simulink model "Thruster_Example_rw"  (R2024b)
settings: Solver=ode4  StartTime=0.0  StopTime=2000  FixedStep=0.01  RelTol=1e-3
undefined symbols (not defined in the file): Cube_L, dt, F_vec, Iws, M_rw, m_tot, norm_Ib, Omega1_init, Omega2_init, Omega3_init, Omega4_init, qb0, rad2rpm, RCS_F, RCS_F_vec, RCS_Pos, RCS_pos, RCS_PWM_Freq, RCS_Sampling_time, RCS_THR_vec, REL_TS_POS_I_0, REL_TS_VEL_I_0, RW_As, RW_Max_Speed, RW_Omegad_max, sat, SC_Ib, SC_state0, SS_Total_Mass, TC_Kepler, THR_dt, THR_Force, THR_freq, THR_Pos, TS_Ib, TS_qb0, TS_state0, TS_wb0, wb0, X, Y, Z
libraries: sm_lib x348, nesl_utility x236, simulink_extras x115, sharedtransform x64, aerolibutil x38, simulink x28, sharedutil x13
(part 4 of 16)

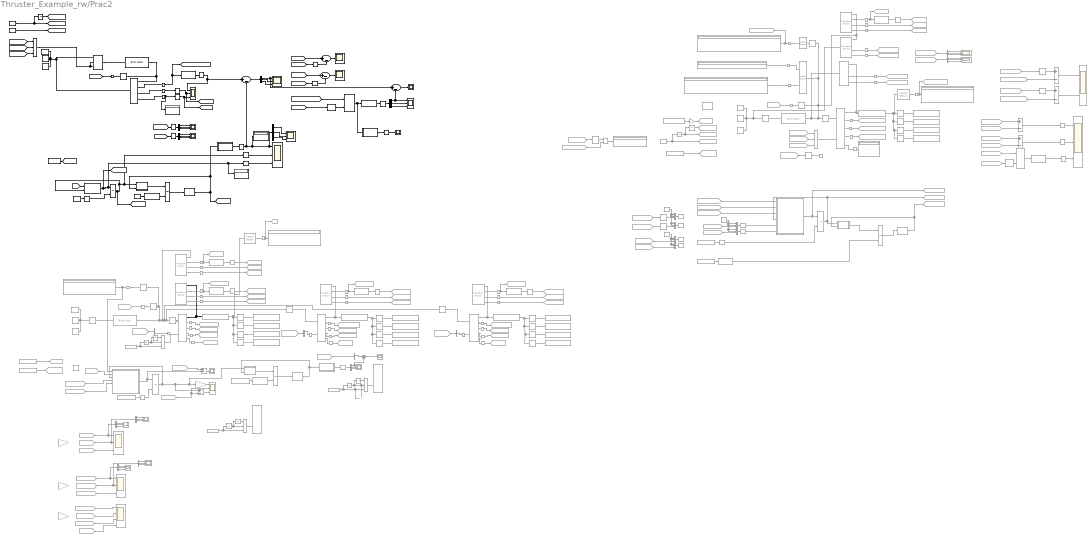
== system Thruster_Example_rw/Prac2 ==
  note: inertia sensor 써야 wheel까지 포함한 MOI 구해짐.
      | 여기서 구해진 MOI를 사용해야 오차가 없다.
  note: 이렇게 하면, wheel의 각가속도, 각속도 다 계산 안해도 넣어진다.
  (rad/sec) to RPM{,1,3..4} (4 alike) : Gain  Commented=on  Gain=60/(2*pi)
  6-DOF Joint : sm_lib/Joints/6-DOF Joint  Commented=on  JointMode=Normal  SenseConstraintForce=off  SenseConstraintForceX=off  SenseConstraintForceY=off  SenseConstraintForceZ=off  SenseConstraintTorque=off  SenseConstraintTorqueX=off  SenseConstraintTorqueY=off  SenseConstraintTorqueZ=off  SenseTotalForce=off  SenseTotalForceX=off  SenseTotalForceY=off  SenseTotalForceZ=off  SenseTotalTorque=off  SenseTotalTorqueX=off  SenseTotalTorqueY=off  SenseTotalTorqueZ=off  CompositeWrenchDir=FollowerOnBase  CompositeWrenchFrame=BaseFrame  PxEquilibriumPosition=0  PxEquilibriumPositionUnits=m  PxSpringStiffness=0  PxSpringStiffnessUnits=N/m  PxDampingCoefficient=0  PxDampingCoefficientUnits=N/(m/s)  PxTorqueActuationMode=NoTorque  PxMotionActuationMode=ComputedMotion  PxSensePosition=off  PxSenseVelocity=off  PxSenseAcceleration=off  PxSenseTorqueForce=off  PxSenseLowerLimitTorqueForce=off  PxSenseUpperLimitTorqueForce=off  PxLowerLimitSpecify=off  PxLowerLimitBound=-1  PxLowerLimitBoundUnits=m  PxLowerLimitStiffness=1e6  PxLowerLimitStiffnessUnits=N/m  PxLowerLimitDamping=1e3  PxLowerLimitDampingUnits=N/(m/s)  PxLowerLimitTransitionRegionWidth=1e-4  PxLowerLimitTransitionRegionWidthUnits=m  PxUpperLimitSpecify=off  PxUpperLimitBound=1  PxUpperLimitBoundUnits=m  PxUpperLimitStiffness=1e6  PxUpperLimitStiffnessUnits=N/m  PxUpperLimitDamping=1e3  PxUpperLimitDampingUnits=N/(m/s)  PxUpperLimitTransitionRegionWidth=1e-4  PxUpperLimitTransitionRegionWidthUnits=m  PxPositionTargetSpecify=off  PxPositionTargetPriority=High  PxPositionTargetValue=0  PxPositionTargetValueUnits=m  PxVelocityTargetSpecify=off  PxVelocityTargetPriority=High  PxVelocityTargetValue=0  PxVelocityTargetValueUnits=m/s  PyEquilibriumPosition=0  PyEquilibriumPositionUnits=m  PySpringStiffness=0  PySpringStiffnessUnits=N/m  PyDampingCoefficient=0  PyDampingCoefficientUnits=N/(m/s)  PyTorqueActuationMode=NoTorque  PyMotionActuationMode=ComputedMotion  PySensePosition=off  PySenseVelocity=off  PySenseAcceleration=off  PySenseTorqueForce=off  PySenseLowerLimitTorqueForce=off  PySenseUpperLimitTorqueForce=off  PyLowerLimitSpecify=off  PyLowerLimitBound=-1  PyLowerLimitBoundUnits=m  PyLowerLimitStiffness=1e6  PyLowerLimitStiffnessUnits=N/m  PyLowerLimitDamping=1e3  PyLowerLimitDampingUnits=N/(m/s)  PyLowerLimitTransitionRegionWidth=1e-4  PyLowerLimitTransitionRegionWidthUnits=m  PyUpperLimitSpecify=off  PyUpperLimitBound=1  PyUpperLimitBoundUnits=m  PyUpperLimitStiffness=1e6  PyUpperLimitStiffnessUnits=N/m  PyUpperLimitDamping=1e3  PyUpperLimitDampingUnits=N/(m/s)  PyUpperLimitTransitionRegionWidth=1e-4  PyUpperLimitTransitionRegionWidthUnits=m  PyPositionTargetSpecify=off  PyPositionTargetPriority=High  PyPositionTargetValue=0  PyPositionTargetValueUnits=m  PyVelocityTargetSpecify=off  PyVelocityTargetPriority=High  PyVelocityTargetValue=0  PyVelocityTargetValueUnits=m/s  PzEquilibriumPosition=0  PzEquilibriumPositionUnits=m  PzSpringStiffness=0  PzSpringStiffnessUnits=N/m  PzDampingCoefficient=0  PzDampingCoefficientUnits=N/(m/s)  PzTorqueActuationMode=NoTorque  PzMotionActuationMode=ComputedMotion  PzSensePosition=off  PzSenseVelocity=off  PzSenseAcceleration=off  PzSenseTorqueForce=off  PzSenseLowerLimitTorqueForce=off  PzSenseUpperLimitTorqueForce=off  PzLowerLimitSpecify=off  PzLowerLimitBound=-1  PzLowerLimitBoundUnits=m  PzLowerLimitStiffness=1e6  PzLowerLimitStiffnessUnits=N/m  PzLowerLimitDamping=1e3  PzLowerLimitDampingUnits=N/(m/s)  PzLowerLimitTransitionRegionWidth=1e-4  PzLowerLimitTransitionRegionWidthUnits=m  PzUpperLimitSpecify=off  PzUpperLimitBound=1  PzUpperLimitBoundUnits=m  PzUpperLimitStiffness=1e6  PzUpperLimitStiffnessUnits=N/m  PzUpperLimitDamping=1e3  PzUpperLimitDampingUnits=N/(m/s)  PzUpperLimitTransitionRegionWidth=1e-4  PzUpperLimitTransitionRegionWidthUnits=m  PzPositionTargetSpecify=off  PzPositionTargetPriority=High  PzPositionTargetValue=0  PzPositionTargetValueUnits=m  PzVelocityTargetSpecify=off  PzVelocityTargetPriority=High  PzVelocityTargetValue=0  PzVelocityTargetValueUnits=m/s  SphEqPosRotationMethod=None  SphEqPosRotationAngleUnits=deg  SphEqPosRotationStandardAxis=+Z  SphEqPosRotationAngle=0.0  SphEqPosRotationArbitraryAxis=[0 0 1]  SphEqPosFollAlignAxisA=+X  SphEqPosBaseAlignAxisA=+Y  SphEqPosFollAlignAxisB=+Y  SphEqPosBaseAlignAxisB=+Z  SphEqPosRotationSequenceAxes=FollowerAxes  SphEqPosRotationSequence=XYX  SphEqPosRotationSequenceAngles=[0 0 0]  SphEqPosRotationSequenceAnglesUnits=deg  SphEqPosRotationMatrix=[1 0 0; 0 1 0; 0 0 1]  SphEqPosQuaternion=[1 0 0 0]  SphSpringStiffness=0  SphSpringStiffnessUnits=N*m/deg  SphDampingCoefficient=0  SphDampingCoefficientUnits=N*m/(deg/s)  SphActuateTorqueX=off  SphActuateTorqueY=off  SphActuateTorqueZ=on  SphActuateTorque=off  SphTorqueActuationMode=NoTorque  SphMotionActuationMode=ComputedMotion  SphActuationFrame=BaseFrame  SphSensePosition=off  SphSenseVelocityX=off  SphSenseVelocityY=off  SphSenseVelocityZ=off  SphSenseVelocity=off  SphSenseAccelerationX=off  SphSenseAccelerationY=off  SphSenseAccelerationZ=off  SphSenseAcceleration=off  SphSenseTorqueX=off  SphSenseTorqueY=off  SphSenseTorqueZ=off  SphSenseTorqueForce=off  SphSenseLowerLimitTorqueMag=off  SphSenseUpperLimitTorqueMag=off  SphSensingFrame=BaseFrame  SphLowerLimitSpecify=off  SphLowerLimitBound=15  SphLowerLimitBoundUnits=deg  SphLowerLimitStiffness=1e4  SphLowerLimitStiffnessUnits=N*m/deg  SphLowerLimitDamping=10  SphLowerLimitDampingUnits=N*m/(deg/s)  SphLowerLimitTransitionRegionWidth=0.1  SphLowerLimitTransitionRegionWidthUnits=deg  SphUpperLimitSpecify=off  SphUpperLimitBound=45  SphUpperLimitBoundUnits=deg  SphUpperLimitStiffness=1e4  SphUpperLimitStiffnessUnits=N*m/deg  SphUpperLimitDamping=10  SphUpperLimitDampingUnits=N*m/(deg/s)  SphUpperLimitTransitionRegionWidth=0.1  SphUpperLimitTransitionRegionWidthUnits=deg  SphPositionTargetRotationMethod=None  SphPositionTargetRotationAngleUnits=deg  SphPositionTargetRotationStandardAxis=+Z  SphPositionTargetRotationAngle=0.0  SphPositionTargetRotationArbitraryAxis=[0 0 1]  SphPositionTargetFollAlignAxisA=+X  SphPositionTargetBaseAlignAxisA=+Y  SphPositionTargetFollAlignAxisB=+Y  SphPositionTargetBaseAlignAxisB=+Z  SphPositionTargetRotationSequenceAxes=FollowerAxes  SphPositionTargetRotationSequence=XYX  SphPositionTargetRotationSequenceAngles=[0 0 0]  SphPositionTargetRotationSequenceAnglesUnits=deg  SphPositionTargetRotationMatrix=[1 0 0; 0 1 0; 0 0 1]  SphPositionTargetQuaternion=[1 0 0 0]  SphPositionTargetSpecify=off  SphPositionTargetPriority=High  SphVelocityTargetValue=[0 0 0]  SphVelocityTargetValueUnits=deg/s  SphVelocityTargetSpecify=off  SphVelocityTargetPriority=High  SphVelocityTargetInFollowerFrame=on
  6-DOF Joint2 : sm_lib/Joints/6-DOF Joint  Commented=on  JointMode=Normal  SenseConstraintForce=off  SenseConstraintForceX=off  SenseConstraintForceY=off  SenseConstraintForceZ=off  SenseConstraintTorque=off  SenseConstraintTorqueX=off  SenseConstraintTorqueY=off  SenseConstraintTorqueZ=off  SenseTotalForce=off  SenseTotalForceX=off  SenseTotalForceY=off  SenseTotalForceZ=off  SenseTotalTorque=off  SenseTotalTorqueX=off  SenseTotalTorqueY=off  SenseTotalTorqueZ=off  CompositeWrenchDir=FollowerOnBase  CompositeWrenchFrame=BaseFrame  PxEquilibriumPosition=0  PxEquilibriumPositionUnits=m  PxSpringStiffness=0  PxSpringStiffnessUnits=N/m  PxDampingCoefficient=0  PxDampingCoefficientUnits=N/(m/s)  PxTorqueActuationMode=NoTorque  PxMotionActuationMode=ComputedMotion  PxSensePosition=off  PxSenseVelocity=off  PxSenseAcceleration=off  PxSenseTorqueForce=off  PxSenseLowerLimitTorqueForce=off  PxSenseUpperLimitTorqueForce=off  PxLowerLimitSpecify=off  PxLowerLimitBound=-1  PxLowerLimitBoundUnits=m  PxLowerLimitStiffness=1e6  PxLowerLimitStiffnessUnits=N/m  PxLowerLimitDamping=1e3  PxLowerLimitDampingUnits=N/(m/s)  PxLowerLimitTransitionRegionWidth=1e-4  PxLowerLimitTransitionRegionWidthUnits=m  PxUpperLimitSpecify=off  PxUpperLimitBound=1  PxUpperLimitBoundUnits=m  PxUpperLimitStiffness=1e6  PxUpperLimitStiffnessUnits=N/m  PxUpperLimitDamping=1e3  PxUpperLimitDampingUnits=N/(m/s)  PxUpperLimitTransitionRegionWidth=1e-4  PxUpperLimitTransitionRegionWidthUnits=m  PxPositionTargetSpecify=off  PxPositionTargetPriority=High  PxPositionTargetValue=0  PxPositionTargetValueUnits=m  PxVelocityTargetSpecify=off  PxVelocityTargetPriority=High  PxVelocityTargetValue=0  PxVelocityTargetValueUnits=m/s  PyEquilibriumPosition=0  PyEquilibriumPositionUnits=m  PySpringStiffness=0  PySpringStiffnessUnits=N/m  PyDampingCoefficient=0  PyDampingCoefficientUnits=N/(m/s)  PyTorqueActuationMode=NoTorque  PyMotionActuationMode=ComputedMotion  PySensePosition=off  PySenseVelocity=off  PySenseAcceleration=off  PySenseTorqueForce=off  PySenseLowerLimitTorqueForce=off  PySenseUpperLimitTorqueForce=off  PyLowerLimitSpecify=off  PyLowerLimitBound=-1  PyLowerLimitBoundUnits=m  PyLowerLimitStiffness=1e6  PyLowerLimitStiffnessUnits=N/m  PyLowerLimitDamping=1e3  PyLowerLimitDampingUnits=N/(m/s)  PyLowerLimitTransitionRegionWidth=1e-4  PyLowerLimitTransitionRegionWidthUnits=m  PyUpperLimitSpecify=off  PyUpperLimitBound=1  PyUpperLimitBoundUnits=m  PyUpperLimitStiffness=1e6  PyUpperLimitStiffnessUnits=N/m  PyUpperLimitDamping=1e3  PyUpperLimitDampingUnits=N/(m/s)  PyUpperLimitTransitionRegionWidth=1e-4  PyUpperLimitTransitionRegionWidthUnits=m  PyPositionTargetSpecify=off  PyPositionTargetPriority=High  PyPositionTargetValue=0  PyPositionTargetValueUnits=m  PyVelocityTargetSpecify=off  PyVelocityTargetPriority=High  PyVelocityTargetValue=0  PyVelocityTargetValueUnits=m/s  PzEquilibriumPosition=0  PzEquilibriumPositionUnits=m  PzSpringStiffness=0  PzSpringStiffnessUnits=N/m  PzDampingCoefficient=0  PzDampingCoefficientUnits=N/(m/s)  PzTorqueActuationMode=NoTorque  PzMotionActuationMode=ComputedMotion  PzSensePosition=off  PzSenseVelocity=off  PzSenseAcceleration=off  PzSenseTorqueForce=off  PzSenseLowerLimitTorqueForce=off  PzSenseUpperLimitTorqueForce=off  PzLowerLimitSpecify=off  PzLowerLimitBound=-1  PzLowerLimitBoundUnits=m  PzLowerLimitStiffness=1e6  PzLowerLimitStiffnessUnits=N/m  PzLowerLimitDamping=1e3  PzLowerLimitDampingUnits=N/(m/s)  PzLowerLimitTransitionRegionWidth=1e-4  PzLowerLimitTransitionRegionWidthUnits=m  PzUpperLimitSpecify=off  PzUpperLimitBound=1  PzUpperLimitBoundUnits=m  PzUpperLimitStiffness=1e6  PzUpperLimitStiffnessUnits=N/m  PzUpperLimitDamping=1e3  PzUpperLimitDampingUnits=N/(m/s)  PzUpperLimitTransitionRegionWidth=1e-4  PzUpperLimitTransitionRegionWidthUnits=m  PzPositionTargetSpecify=off  PzPositionTargetPriority=High  PzPositionTargetValue=0  PzPositionTargetValueUnits=m  PzVelocityTargetSpecify=off  PzVelocityTargetPriority=High  PzVelocityTargetValue=0  PzVelocityTargetValueUnits=m/s  SphEqPosRotationMethod=None  SphEqPosRotationAngleUnits=deg  SphEqPosRotationStandardAxis=+Z  SphEqPosRotationAngle=0.0  SphEqPosRotationArbitraryAxis=[0 0 1]  SphEqPosFollAlignAxisA=+X  SphEqPosBaseAlignAxisA=+Y  SphEqPosFollAlignAxisB=+Y  SphEqPosBaseAlignAxisB=+Z  SphEqPosRotationSequenceAxes=FollowerAxes  SphEqPosRotationSequence=XYX  SphEqPosRotationSequenceAngles=[0 0 0]  SphEqPosRotationSequenceAnglesUnits=deg  SphEqPosRotationMatrix=[1 0 0; 0 1 0; 0 0 1]  SphEqPosQuaternion=[1 0 0 0]  SphSpringStiffness=0  SphSpringStiffnessUnits=N*m/deg  SphDampingCoefficient=0  SphDampingCoefficientUnits=N*m/(deg/s)  SphActuateTorqueX=off  SphActuateTorqueY=off  SphActuateTorqueZ=on  SphActuateTorque=off  SphTorqueActuationMode=NoTorque  SphMotionActuationMode=ComputedMotion  SphActuationFrame=BaseFrame  SphSensePosition=off  SphSenseVelocityX=off  SphSenseVelocityY=off  SphSenseVelocityZ=off  SphSenseVelocity=off  SphSenseAccelerationX=off  SphSenseAccelerationY=off  SphSenseAccelerationZ=off  SphSenseAcceleration=off  SphSenseTorqueX=off  SphSenseTorqueY=off  SphSenseTorqueZ=off  SphSenseTorqueForce=off  SphSenseLowerLimitTorqueMag=off  SphSenseUpperLimitTorqueMag=off  SphSensingFrame=BaseFrame  SphLowerLimitSpecify=off  SphLowerLimitBound=15  SphLowerLimitBoundUnits=deg  SphLowerLimitStiffness=1e4  SphLowerLimitStiffnessUnits=N*m/deg  SphLowerLimitDamping=10  SphLowerLimitDampingUnits=N*m/(deg/s)  SphLowerLimitTransitionRegionWidth=0.1  SphLowerLimitTransitionRegionWidthUnits=deg  SphUpperLimitSpecify=off  SphUpperLimitBound=45  SphUpperLimitBoundUnits=deg  SphUpperLimitStiffness=1e4  SphUpperLimitStiffnessUnits=N*m/deg  SphUpperLimitDamping=10  SphUpperLimitDampingUnits=N*m/(deg/s)  SphUpperLimitTransitionRegionWidth=0.1  SphUpperLimitTransitionRegionWidthUnits=deg  SphPositionTargetRotationMethod=None  SphPositionTargetRotationAngleUnits=deg  SphPositionTargetRotationStandardAxis=+Z  SphPositionTargetRotationAngle=0.0  SphPositionTargetRotationArbitraryAxis=[0 0 1]  SphPositionTargetFollAlignAxisA=+X  SphPositionTargetBaseAlignAxisA=+Y  SphPositionTargetFollAlignAxisB=+Y  SphPositionTargetBaseAlignAxisB=+Z  SphPositionTargetRotationSequenceAxes=FollowerAxes  SphPositionTargetRotationSequence=XYX  SphPositionTargetRotationSequenceAngles=[0 0 0]  SphPositionTargetRotationSequenceAnglesUnits=deg  SphPositionTargetRotationMatrix=[1 0 0; 0 1 0; 0 0 1]  SphPositionTargetQuaternion=[1 0 0 0]  SphPositionTargetSpecify=off  SphPositionTargetPriority=High  SphVelocityTargetValue=[0 0 0]  SphVelocityTargetValueUnits=deg/s  SphVelocityTargetSpecify=off  SphVelocityTargetPriority=High  SphVelocityTargetInFollowerFrame=on
  Add{,1..5} (6 alike) : Sum  Commented=on  Inputs=+-
  Base : sm_lib/Body Elements/Brick Solid  GraphicAmbientColor=[0.15 0.15 0.15 1.0]  BasedOnType=Mass  BrickDimensions=[0.3 0.3 0.3]  BrickDimensionsUnits=m  CenterOfMass=[0 0 0]  CenterOfMassUnits=m  GraphicDiffuseColor=[0.0 0.8 0.8]  Density=1000  DensityUnits=kg/m^3  DoExposeReferenceFrame=on  GraphicEmissiveColor=[0.0 0.0 0.0 1.0]  ExportEntireGeometry=off  SerializedFrames=<Frames><Frame><Id>Frame1</Id><Value><Name>CM_F</Name><Origin><Source>CenterOfMassFrame</Source><FeatureName></FeatureName></Origin><PrimaryAxis><DefinedDirection>+Z</DefinedDirection><Source>ReferenceFrame</Source><SourceDirection>+Z</SourceDirection><FeatureName></FeatureName></PrimaryAxis><SecondaryAxis><DefinedDirection>+X</DefinedDirection><Source>ReferenceFrame</Source><SourceDirection>+X</SourceDirection><FeatureName></FeatureName></SecondaryAxis></Value></Frame></Frames>  MarkerShape=Sphere  MarkerSize=10  GraphicType=FromGeometry  InertiaType=CalculateFromGeometry  Mass=10  MassUnits=kg  MomentsOfInertia=[1 1 1]  MomentsOfInertiaUnits=kg*m^2  GraphicOpacity=1  ProductsOfInertia=[0 0 0]  ProductsOfInertiaUnits=kg*m^2  GraphicShininess=75  GraphicSpecularColor=[0.5 0.5 0.5 1.0]  GraphicVisPropType=SimpleVisualProperties
  Base1 : sm_lib/Body Elements/Brick Solid  Commented=on  GraphicAmbientColor=[0.15 0.15 0.15 1.0]  BasedOnType=Mass  BrickDimensions=[Cube_L Cube_L Cube_L]  BrickDimensionsUnits=m  CenterOfMass=[0 0 0]  CenterOfMassUnits=m  GraphicDiffuseColor=[0.0 0.8 0.8]  Density=1000  DensityUnits=kg/m^3  DoExposeReferenceFrame=on  GraphicEmissiveColor=[0.0 0.0 0.0 1.0]  ExportEntireGeometry=off  SerializedFrames=<Frames><Frame><Id>Frame1</Id><Value><Name>CM_F</Name><Origin><Source>CenterOfMassFrame</Source><FeatureName></FeatureName></Origin><PrimaryAxis><DefinedDirection>+Z</DefinedDirection><Source>ReferenceFrame</Source><SourceDirection>+Z</SourceDirection><FeatureName></FeatureName></PrimaryAxis><SecondaryAxis><DefinedDirection>+X</DefinedDirection><Source>ReferenceFrame</Source><SourceDirection>+X</SourceDirection><FeatureName></FeatureName></SecondaryAxis></Value></Frame></Frames>  MarkerShape=Sphere  MarkerSize=10  GraphicType=FromGeometry  InertiaType=CalculateFromGeometry  Mass=10  MassUnits=kg  MomentsOfInertia=[1 1 1]  MomentsOfInertiaUnits=kg*m^2  GraphicOpacity=0.2  ProductsOfInertia=[0 0 0]  ProductsOfInertiaUnits=kg*m^2  GraphicShininess=75  GraphicSpecularColor=[0.5 0.5 0.5 1.0]  GraphicVisPropType=SimpleVisualProperties
  Base2 : sm_lib/Body Elements/Brick Solid  Commented=on  GraphicAmbientColor=[0.15 0.15 0.15 1.0]  BasedOnType=Mass  BrickDimensions=[0.3 0.3 0.3]  BrickDimensionsUnits=m  CenterOfMass=[0 0 0]  CenterOfMassUnits=m  GraphicDiffuseColor=[0.0 0.8 0.8]  Density=1000  DensityUnits=kg/m^3  DoExposeReferenceFrame=on  GraphicEmissiveColor=[0.0 0.0 0.0 1.0]  ExportEntireGeometry=off  SerializedFrames=<Frames><Frame><Id>Frame1</Id><Value><Name>CM_F</Name><Origin><Source>CenterOfMassFrame</Source><FeatureName></FeatureName></Origin><PrimaryAxis><DefinedDirection>+Z</DefinedDirection><Source>ReferenceFrame</Source><SourceDirection>+Z</SourceDirection><FeatureName></FeatureName></PrimaryAxis><SecondaryAxis><DefinedDirection>+X</DefinedDirection><Source>ReferenceFrame</Source><SourceDirection>+X</SourceDirection><FeatureName></FeatureName></SecondaryAxis></Value></Frame></Frames>  MarkerShape=Sphere  MarkerSize=10  GraphicType=FromGeometry  InertiaType=CalculateFromGeometry  Mass=10  MassUnits=kg  MomentsOfInertia=[1 1 1]  MomentsOfInertiaUnits=kg*m^2  GraphicOpacity=0.2  ProductsOfInertia=[0 0 0]  ProductsOfInertiaUnits=kg*m^2  GraphicShininess=75  GraphicSpecularColor=[0.5 0.5 0.5 1.0]  GraphicVisPropType=SimpleVisualProperties
  Constant : Constant  Commented=on  Value=0
  Constant1 : Constant  Value=[0 0 0]
  Constant10 : Constant  Commented=on  Value=0.001
  Constant11 : Constant  Commented=on  Value=0.001
  Constant12 : Constant  Commented=on  Value=0
  Constant13 : Constant  Commented=on  Value=0
  Constant14 : Constant  Commented=on  Value=[0.0025 0 0.0025]
  Constant15 : Constant  Commented=on  Value=[0 0 -0.0025]
  Constant{7,9,16..17} (4 alike) : Constant  Commented=on  Value=[0 0 0]
  Constant2 : Constant  Value=[0 0 0]
  Constant3 : Constant  Value=[0 0 0]
  Constant4 : Constant  Commented=on  Value=sat
  Constant5 : Constant  Commented=on  Value=[0.25 0 0.25]
  Constant6 : Constant  Commented=on  Value=[0.25 0 -0.25]
  Constant8 : Constant  Commented=on  Value=0.001
  Degrees to Radians : simulink_extras/Transformations/Degrees to Radians
  Degrees to Radians1 : simulink_extras/Transformations/Degrees to Radians  Commented=on
  Degrees to Radians2 : simulink_extras/Transformations/Degrees to Radians  Commented=on
  Degrees to Radians3 : simulink_extras/Transformations/Degrees to Radians
  Degrees to Radians4 : simulink_extras/Transformations/Degrees to Radians
  Demux{,1..2,11..12} (5 alike) : Demux  Outputs=3
  Demux{3..10,23..25} (11 alike) : Demux  Commented=on  Outputs=3
  Display : Display
  Display1 : Display
  Display{3..10} (8 alike) : Display  Commented=on
  Display2 : Display
  Divide : Product  Commented=on  Inputs=*/
  "ERROR : Wd, W, Quat" : Scope  Commented=on  NumInputPorts=3
  External Force and Torque : sm_lib/Forces and Torques/External Force and Torque  ForceResolutionFrame=AttachedFrame  EnableForceX=off  EnableForceY=off  EnableForceZ=off  EnableForce=off  TorqueResolutionFrame=World  EnableTorqueX=off  EnableTorqueY=off  EnableTorqueZ=off  EnableTorque=on
  External Force and Torque1 : sm_lib/Forces and Torques/External Force and Torque  Commented=on  ForceResolutionFrame=World  EnableForceX=off  EnableForceY=off  EnableForceZ=off  EnableForce=off  TorqueResolutionFrame=AttachedFrame  EnableTorqueX=off  EnableTorqueY=off  EnableTorqueZ=off  EnableTorque=on
  External Force and Torque2 : sm_lib/Forces and Torques/External Force and Torque  Commented=on  ForceResolutionFrame=World  EnableForceX=off  EnableForceY=off  EnableForceZ=off  EnableForce=off  TorqueResolutionFrame=AttachedFrame  EnableTorqueX=off  EnableTorqueY=off  EnableTorqueZ=off  EnableTorque=on
  Fly_Wheel : sm_lib/Body Elements/Cylindrical Solid  Commented=on  GraphicAmbientColor=[0.15 0.15 0.15 1.0]  BasedOnType=Mass  CenterOfMass=[0 0 0]  CenterOfMassUnits=m  GraphicDiffuseColor=[0.0 0.0 1.0]  CylinderLength=0.01  CylinderLengthUnits=m  CylinderRadius=0.015  CylinderRadiusUnits=m  Density=1000  DensityUnits=kg/m^3  DoExposeReferenceFrame=on  GraphicEmissiveColor=[0.0 0.0 0.0 1.0]  ExportEntireGeometry=off  SerializedFrames=<Frames><Frame><Id>Frame1</Id><Value><Name>Sticker_F</Name><Origin><Source>GeometricFeature</Source><FeatureName>top surface</FeatureName></Origin><PrimaryAxis><DefinedDirection>+Z</DefinedDirection><Source>ReferenceFrame</Source><SourceDirection>+Z</SourceDirection><FeatureName></FeatureName></PrimaryAxis><SecondaryAxis><DefinedDirection>+X</DefinedDirection><Source>ReferenceFrame</Source><SourceDirection>+X</SourceDirection><FeatureName></FeatureName></SecondaryAxis></Value></Frame></Frames>  MarkerShape=Sphere  MarkerSize=10  GraphicType=FromGeometry  InertiaType=CalculateFromGeometry  Mass=10  MassUnits=kg  MomentsOfInertia=[1 1 1]  MomentsOfInertiaUnits=kg*m^2  GraphicOpacity=1.0  ProductsOfInertia=[0 0 0]  ProductsOfInertiaUnits=kg*m^2  GraphicShininess=75  GraphicSpecularColor=[0.5 0.5 0.5 1.0]  GraphicVisPropType=SimpleVisualProperties
  Fly_Wheel_X : sm_lib/Body Elements/Cylindrical Solid  Commented=on  GraphicAmbientColor=[0.15 0.15 0.15 1.0]  BasedOnType=Mass  CenterOfMass=[0 0 0]  CenterOfMassUnits=m  GraphicDiffuseColor=[1.0 0.0 0]  CylinderLength=L_rw  CylinderLengthUnits=m  CylinderRadius=R_rw  CylinderRadiusUnits=m  Density=1000  DensityUnits=kg/m^3  DoExposeReferenceFrame=on  GraphicEmissiveColor=[0.0 0.0 0.0 1.0]  ExportEntireGeometry=off  SerializedFrames=<Frames><Frame><Id>Frame1</Id><Value><Name>Sticker_F</Name><Origin><Source>GeometricFeature</Source><FeatureName>top surface</FeatureName></Origin><PrimaryAxis><DefinedDirection>+Z</DefinedDirection><Source>ReferenceFrame</Source><SourceDirection>+Z</SourceDirection><FeatureName></FeatureName></PrimaryAxis><SecondaryAxis><DefinedDirection>+X</DefinedDirection><Source>ReferenceFrame</Source><SourceDirection>+X</SourceDirection><FeatureName></FeatureName></SecondaryAxis></Value></Frame></Frames>  MarkerShape=Sphere  MarkerSize=10  GraphicType=FromGeometry  InertiaType=CalculateFromGeometry  Mass=M_rw  MassUnits=kg  MomentsOfInertia=[1 1 1]  MomentsOfInertiaUnits=kg*m^2  GraphicOpacity=1.0  ProductsOfInertia=[0 0 0]  ProductsOfInertiaUnits=kg*m^2  GraphicShininess=75  GraphicSpecularColor=[0.5 0.5 0.5 1.0]  GraphicVisPropType=SimpleVisualProperties
  Fly_Wheel_Y : sm_lib/Body Elements/Cylindrical Solid  Commented=on  GraphicAmbientColor=[0.15 0.15 0.15 1.0]  BasedOnType=Mass  CenterOfMass=[0 0 0]  CenterOfMassUnits=m  GraphicDiffuseColor=[0 1 0]  CylinderLength=L_rw  CylinderLengthUnits=m  CylinderRadius=R_rw  CylinderRadiusUnits=m  Density=1000  DensityUnits=kg/m^3  DoExposeReferenceFrame=on  GraphicEmissiveColor=[0.0 0.0 0.0 1.0]  ExportEntireGeometry=off  SerializedFrames=<Frames><Frame><Id>Frame1</Id><Value><Name>Sticker_F</Name><Origin><Source>GeometricFeature</Source><FeatureName>top surface</FeatureName></Origin><PrimaryAxis><DefinedDirection>+Z</DefinedDirection><Source>ReferenceFrame</Source><SourceDirection>+Z</SourceDirection><FeatureName></FeatureName></PrimaryAxis><SecondaryAxis><DefinedDirection>+X</DefinedDirection><Source>ReferenceFrame</Source><SourceDirection>+X</SourceDirection><FeatureName></FeatureName></SecondaryAxis></Value></Frame></Frames>  MarkerShape=Sphere  MarkerSize=10  GraphicType=FromGeometry  InertiaType=CalculateFromGeometry  Mass=M_rw  MassUnits=kg  MomentsOfInertia=[1 1 1]  MomentsOfInertiaUnits=kg*m^2  GraphicOpacity=1.0  ProductsOfInertia=[0 0 0]  ProductsOfInertiaUnits=kg*m^2  GraphicShininess=75  GraphicSpecularColor=[0.5 0.5 0.5 1.0]  GraphicVisPropType=SimpleVisualProperties
  Fly_Wheel_Z : sm_lib/Body Elements/Cylindrical Solid  Commented=on  GraphicAmbientColor=[0.15 0.15 0.15 1.0]  BasedOnType=Mass  CenterOfMass=[0 0 0]  CenterOfMassUnits=m  GraphicDiffuseColor=[0.0 0.0 1.0]  CylinderLength=L_rw  CylinderLengthUnits=m  CylinderRadius=R_rw  CylinderRadiusUnits=m  Density=1000  DensityUnits=kg/m^3  DoExposeReferenceFrame=on  GraphicEmissiveColor=[0.0 0.0 0.0 1.0]  ExportEntireGeometry=off  SerializedFrames=<Frames><Frame><Id>Frame1</Id><Value><Name>Sticker_F</Name><Origin><Source>GeometricFeature</Source><FeatureName>top surface</FeatureName></Origin><PrimaryAxis><DefinedDirection>+Z</DefinedDirection><Source>ReferenceFrame</Source><SourceDirection>+Z</SourceDirection><FeatureName></FeatureName></PrimaryAxis><SecondaryAxis><DefinedDirection>+X</DefinedDirection><Source>ReferenceFrame</Source><SourceDirection>+X</SourceDirection><FeatureName></FeatureName></SecondaryAxis></Value></Frame></Frames>  MarkerShape=Sphere  MarkerSize=10  GraphicType=FromGeometry  InertiaType=CalculateFromGeometry  Mass=M_rw  MassUnits=kg  MomentsOfInertia=[1 1 1]  MomentsOfInertiaUnits=kg*m^2  GraphicOpacity=1.0  ProductsOfInertia=[0 0 0]  ProductsOfInertiaUnits=kg*m^2  GraphicShininess=75  GraphicSpecularColor=[0.5 0.5 0.5 1.0]  GraphicVisPropType=SimpleVisualProperties
  From : From  Commented=on  GotoTag=RW_Joint_Rate
  From10 : From  Commented=on  GotoTag=Simscape_wd
  From11 : From  Commented=on  GotoTag=Simscape_torque
  From12 : From  Commented=on  GotoTag=Simscape_angle
  From{13..15,34} (4 alike) : From  Commented=on  GotoTag=control_input_Torque
  From16 : From  Commented=on  GotoTag=Revolute_Joint_RW_angle
  From{17,28,32,38,45} (5 alike) : From  Commented=on  GotoTag=Torque_ext
  From18 : From  Commented=on  GotoTag=Revolute_Joint_RW_w
  From19 : From  Commented=on  GotoTag=Revolute_Joint_RW_wd
  From{20,25,43,46} (4 alike) : From  Commented=on  GotoTag=Simscape_RW_w
  From21 : From  Commented=on  GotoTag=Rigid_Body_Eq_w
  From22 : From  Commented=on  GotoTag=Rigid_Body_Eq_q
  From23 : From  Commented=on  GotoTag=Simscape_quat
  From24 : From  Commented=on  GotoTag=Wheel_MOI
  From26 : From  Commented=on  GotoTag=Total_MOI
  From27 : From  Commented=on  GotoTag=Simscape_wb_body
  From29 : From  Commented=on  GotoTag=Simscape_wd_body
  From{30..31,44,47} (4 alike) : From  Commented=on  GotoTag=Simscape_RW_wd
  From33 : From  Commented=on  GotoTag=Total_MOI
  From35 : From  Commented=on  GotoTag=Revolute_Joint_RW_w
  From36 : From  Commented=on  GotoTag=Revolute_Joint_RW_wd
  From37 : From  Commented=on  GotoTag=Revolute_Joint_RW_w
  From39 : From  Commented=on  GotoTag=Simscape_w
  From40 : From  Commented=on  GotoTag=Simscape_wd
  From41 : From  Commented=on  GotoTag=Simscape_angle
  From42 : From  Commented=on  GotoTag=Simscape_RW_angle
  From48 : From  Commented=on  GotoTag=Revolute_Joint_RW_wd
  From49 : From  Commented=on  GotoTag=RW_Joint_Accel
  From50 : From  Commented=on  GotoTag=RW_Joint_Accel
  From51 : From  Commented=on  GotoTag=RW_Joint_Rate
  From52 : From  Commented=on  GotoTag=RW_Joint_Angle
  From53 : From  Commented=on  GotoTag=Rigid_Body_Eq_wd
  From54 : From  Commented=on  GotoTag=Simscape_wb_body
  From55 : From  Commented=on  GotoTag=Simscape_wd_body
  From9 : From  Commented=on  GotoTag=Simscape_w
  Gain : Gain  Commented=on
  Goto{10,24,35,53} (4 alike) : Goto  Commented=on  GotoTag=Revolute_Joint_RW_angle
  Goto{11,17,25,40} (4 alike) : Goto  Commented=on  GotoTag=Simscape_RW_w
  Goto{12,21,26,41} (4 alike) : Goto  Commented=on  GotoTag=Simscape_RW_wd
  Goto13 : Goto  Commented=on  GotoTag=Simscape_RW_angle
  Goto14 : Goto  Commented=on  GotoTag=Simscape_w
  Goto15 : Goto  Commented=on  GotoTag=Simscape_wd
  Goto16 : Goto  Commented=on  GotoTag=Simscape_angle
  Goto18 : Goto  Commented=on  GotoTag=Simscape_quat
  Goto19 : Goto  Commented=on  GotoTag=Simscape_RW_quat
  Goto{20,30,33,48} (4 alike) : Goto  Commented=on  GotoTag=Revolute_Joint_RW_w
  Goto22 : Goto  Commented=on  GotoTag=Simscape_RW_angle
  Goto23 : Goto  Commented=on  GotoTag=Simscape_RW_quat
  Goto27 : Goto  Commented=on  GotoTag=Simscape_RW_angle
  Goto28 : Goto  Commented=on  GotoTag=Simscape_RW_quat
  Goto{7,9,29,39} (4 alike) : Goto  Commented=on  GotoTag=Revolute_Joint_RW_wd
  Goto31 : Goto  Commented=on  GotoTag=Simscape_torque
  Goto32 : Goto  Commented=on  GotoTag=Simscape_torque
  Goto34 : Goto  Commented=on  GotoTag=Torque_ext
  Goto36 : Goto  Commented=on  GotoTag=control_input_Torque
  Goto37 : Goto  Commented=on  GotoTag=Simscape_torque
  Goto38 : Goto  Commented=on  GotoTag=Rigid_Body_Eq_wd
  Goto42 : Goto  Commented=on  GotoTag=control_input_Torque
  Goto43 : Goto  Commented=on  GotoTag=Simscape_w
  Goto44 : Goto  Commented=on  GotoTag=Simscape_wd
  Goto45 : Goto  Commented=on  GotoTag=Simscape_angle
  Goto46 : Goto  Commented=on  GotoTag=Simscape_quat
  Goto47 : Goto  Commented=on  GotoTag=Wheel_MOI
  Goto49 : Goto  Commented=on  GotoTag=Rigid_Body_Eq_w
  Goto50 : Goto  Commented=on  GotoTag=Rigid_Body_Eq_q
  Goto51 : Goto  Commented=on  GotoTag=Total_MOI
  Goto52 : Goto  Commented=on  GotoTag=Torque_ext
  Goto54 : Goto  Commented=on  GotoTag=Simscape_wb_body
  Goto55 : Goto  Commented=on  GotoTag=Simscape_wd_body
  Goto8 : Goto  Commented=on  GotoTag=I_rw
  Inertia Sensor : sm_lib/Body Elements/Inertia Sensor  Commented=on  SensorExtent=Mechanism  SpanWeldJoints=off  ExcludeGroundedBodies=off  MeasurementFrame=Attached  SenseMass=off  SenseCenterOfMass=off  SenseInertiaMatrix=on  SenseCenteredInertiaMatrix=off  SensePrincipalInertiaMatrix=off  SenseRotationMatrix=off  GraphicType=PrincipalInertiaFrame  PrincipalInertiaFrameSize=20  GraphicVisPropType=SimpleVisualProperties  GraphicDiffuseColor=[0.5 0.5 0.5]  GraphicSpecularColor=[0.5 0.5 0.5 1.0]  GraphicAmbientColor=[0.15 0.15 0.15 1.0]  GraphicEmissiveColor=[0.0 0.0 0.0 1.0]  GraphicShininess=75  GraphicOpacity=1.0
  Inertia Sensor1 : sm_lib/Body Elements/Inertia Sensor  Commented=on  SensorExtent=BodyGroup  SpanWeldJoints=off  ExcludeGroundedBodies=off  MeasurementFrame=Attached  SenseMass=off  SenseCenterOfMass=off  SenseInertiaMatrix=on  SenseCenteredInertiaMatrix=off  SensePrincipalInertiaMatrix=off  SenseRotationMatrix=off  GraphicType=PrincipalInertiaFrame  PrincipalInertiaFrameSize=20  GraphicVisPropType=SimpleVisualProperties  GraphicDiffuseColor=[0.5 0.5 0.5]  GraphicSpecularColor=[0.5 0.5 0.5 1.0]  GraphicAmbientColor=[0.15 0.15 0.15 1.0]  GraphicEmissiveColor=[0.0 0.0 0.0 1.0]  GraphicShininess=75  GraphicOpacity=1.0
  Inertia Sensor2 : sm_lib/Body Elements/Inertia Sensor  Commented=on  SensorExtent=Mechanism  SpanWeldJoints=off  ExcludeGroundedBodies=off  MeasurementFrame=Attached  SenseMass=off  SenseCenterOfMass=on  SenseInertiaMatrix=on  SenseCenteredInertiaMatrix=off  SensePrincipalInertiaMatrix=off  SenseRotationMatrix=off  GraphicType=PrincipalInertiaFrame  PrincipalInertiaFrameSize=20  GraphicVisPropType=SimpleVisualProperties  GraphicDiffuseColor=[0.5 0.5 0.5]  GraphicSpecularColor=[0.5 0.5 0.5 1.0]  GraphicAmbientColor=[0.15 0.15 0.15 1.0]  GraphicEmissiveColor=[0.0 0.0 0.0 1.0]  GraphicShininess=75  GraphicOpacity=1.0
  Inertia Sensor3 : sm_lib/Body Elements/Inertia Sensor  Commented=on  SensorExtent=BodyGroup  SpanWeldJoints=off  ExcludeGroundedBodies=off  MeasurementFrame=Attached  SenseMass=off  SenseCenterOfMass=off  SenseInertiaMatrix=on  SenseCenteredInertiaMatrix=off  SensePrincipalInertiaMatrix=off  SenseRotationMatrix=off  GraphicType=PrincipalInertiaFrame  PrincipalInertiaFrameSize=20  GraphicVisPropType=SimpleVisualProperties  GraphicDiffuseColor=[0.5 0.5 0.5]  GraphicSpecularColor=[0.5 0.5 0.5 1.0]  GraphicAmbientColor=[0.15 0.15 0.15 1.0]  GraphicEmissiveColor=[0.0 0.0 0.0 1.0]  GraphicShininess=75  GraphicOpacity=1.0
  Inertia Sensor4 : sm_lib/Body Elements/Inertia Sensor  Commented=on  SensorExtent=Mechanism  SpanWeldJoints=off  ExcludeGroundedBodies=off  MeasurementFrame=Attached  SenseMass=off  SenseCenterOfMass=off  SenseInertiaMatrix=on  SenseCenteredInertiaMatrix=off  SensePrincipalInertiaMatrix=off  SenseRotationMatrix=off  GraphicType=PrincipalInertiaFrame  PrincipalInertiaFrameSize=20  GraphicVisPropType=SimpleVisualProperties  GraphicDiffuseColor=[0.5 0.5 0.5]  GraphicSpecularColor=[0.5 0.5 0.5 1.0]  GraphicAmbientColor=[0.15 0.15 0.15 1.0]  GraphicEmissiveColor=[0.0 0.0 0.0 1.0]  GraphicShininess=75  GraphicOpacity=1.0
  Integrator : Integrator  InitialConditionSource=external
  Integrator1 : Integrator  InitialConditionSource=external
  Integrator{2..3,5..6,8..11} (8 alike) : Integrator  Commented=on
  Integrator{4,7,12..13} (4 alike) : Integrator  Commented=on  InitialConditionSource=external
  Integrator15 : Integrator
  Mechanism Configuration : sm_lib/Utilities/Mechanism Configuration  Commented=on  UniformGravity=None  GravityVector=[0 0 -9.80665]  GravityVectorUnits=m/s^2  LinearizationDelta=0.001  JointModeTransitionNonlinearIterations=2
  Mechanism Configuration1 : sm_lib/Utilities/Mechanism Configuration  UniformGravity=None  GravityVector=[0 0 -9.80665]  GravityVectorUnits=m/s^2  LinearizationDelta=0.001  JointModeTransitionNonlinearIterations=2
  Mechanism Configuration2 : sm_lib/Utilities/Mechanism Configuration  Commented=on  UniformGravity=None  GravityVector=[0 0 -9.80665]  GravityVectorUnits=m/s^2  LinearizationDelta=0.001  JointModeTransitionNonlinearIterations=2
  Mux{,1..5} (6 alike) : Mux  Commented=on  Inputs=3
  PS-Simulink Converter : nesl_utility/PS-Simulink Converter  PhysicalDomain=network_engine_domain  SubClassName=ps_output  LeftPortType=input  RightPortType=output  PseudoPeriodic=off  Frequencies=[]  VectorFormat=inherit  Unit=inherit  AffineConversion=off
  PS-Simulink Converter1 : nesl_utility/PS-Simulink Converter  PhysicalDomain=network_engine_domain  SubClassName=ps_output  LeftPortType=input  RightPortType=output  PseudoPeriodic=off  Frequencies=[]  VectorFormat=inherit  Unit=inherit  AffineConversion=off
  PS-Simulink Converter{3..43} (41 alike) : nesl_utility/PS-Simulink Converter  Commented=on  PhysicalDomain=network_engine_domain  SubClassName=ps_output  LeftPortType=input  RightPortType=output  PseudoPeriodic=off  Frequencies=[]  VectorFormat=inherit  Unit=inherit  AffineConversion=off
  PS-Simulink Converter2 : nesl_utility/PS-Simulink Converter  PhysicalDomain=network_engine_domain  SubClassName=ps_output  LeftPortType=input  RightPortType=output  PseudoPeriodic=off  Frequencies=[]  VectorFormat=inherit  Unit=inherit  AffineConversion=off
  Quaternion Inverse : aerolibutil/Quaternion Inverse
  Quaternion Inverse1 : aerolibutil/Quaternion Inverse  Commented=on
  Quaternion Multiplication : aerolibutil/Quaternion Multiplication
  Quaternion Multiplication1 : aerolibutil/Quaternion Multiplication  Commented=on
  Quaternion Normalize : sharedutil/Quaternion Normalize  aMode=aMode
  Quaternion Normalize1 : sharedutil/Quaternion Normalize  Commented=on  aMode=aMode
  Quaternion Normalize2 : sharedutil/Quaternion Normalize  Commented=on  aMode=aMode
  Quaternions to Rotation Angles : sharedtransform/Quaternions to Rotation Angles  rotationOrder=ZYX  aMode=aMode
  Quaternions to Rotation Angles{1..2,4..7} (6 alike) : sharedtransform/Quaternions to Rotation Angles  Commented=on  rotationOrder=ZYX  aMode=aMode
  Quaternions to Rotation Angles3 : sharedtransform/Quaternions to Rotation Angles  rotationOrder=ZYX  aMode=aMode
  "RW_diff(Sim,Rev) : wd, w" : Scope  Commented=on  NumInputPorts=2
  Radians to Degrees{,1..7,9..10} (10 alike) : simulink_extras/Transformations/Radians to Degrees
  Radians to Degrees{8,11..18} (9 alike) : simulink_extras/Transformations/Radians to Degrees  Commented=on
  Reshape{,1..5} (6 alike) : Reshape  Commented=on  OutputDimensionality=Column vector (2-D)
  Revolute Joint : sm_lib/Joints/Revolute Joint  Commented=on  JointMode=Normal  SenseConstraintForce=off  SenseConstraintForceX=off  SenseConstraintForceY=off  SenseConstraintForceZ=off  SenseConstraintTorque=off  SenseConstraintTorqueX=off  SenseConstraintTorqueY=off  SenseConstraintTorqueZ=off  SenseTotalForce=off  SenseTotalForceX=off  SenseTotalForceY=off  SenseTotalForceZ=off  SenseTotalTorque=off  SenseTotalTorqueX=off  SenseTotalTorqueY=off  SenseTotalTorqueZ=off  CompositeWrenchDir=FollowerOnBase  CompositeWrenchFrame=BaseFrame  EquilibriumPosition=0  EquilibriumPositionUnits=deg  SpringStiffness=0  SpringStiffnessUnits=N*m/deg  DampingCoefficient=0  DampingCoefficientUnits=N*m/(deg/s)  TorqueActuationMode=ComputedTorque  MotionActuationMode=InputMotion  SensePosition=on  SenseVelocity=on  SenseAcceleration=on  SenseTorqueForce=on  SenseLowerLimitTorqueForce=off  SenseUpperLimitTorqueForce=off  LowerLimitSpecify=off  LowerLimitBound=-90  LowerLimitBoundUnits=deg  LowerLimitStiffness=1e4  LowerLimitStiffnessUnits=N*m/deg  LowerLimitDamping=10  LowerLimitDampingUnits=N*m/(deg/s)  LowerLimitTransitionRegionWidth=0.1  LowerLimitTransitionRegionWidthUnits=deg  UpperLimitSpecify=off  UpperLimitBound=90  UpperLimitBoundUnits=deg  UpperLimitStiffness=1e4  UpperLimitStiffnessUnits=N*m/deg  UpperLimitDamping=10  UpperLimitDampingUnits=N*m/(deg/s)  UpperLimitTransitionRegionWidth=0.1  UpperLimitTransitionRegionWidthUnits=deg  PositionTargetSpecify=off  PositionTargetPriority=High  PositionTargetValue=0  PositionTargetValueUnits=deg  VelocityTargetSpecify=off  VelocityTargetPriority=High  VelocityTargetValue=0  VelocityTargetValueUnits=deg/s
  Revolute Joint1 : sm_lib/Joints/Revolute Joint  Commented=on  JointMode=Normal  SenseConstraintForce=off  SenseConstraintForceX=off  SenseConstraintForceY=off  SenseConstraintForceZ=off  SenseConstraintTorque=off  SenseConstraintTorqueX=off  SenseConstraintTorqueY=off  SenseConstraintTorqueZ=off  SenseTotalForce=off  SenseTotalForceX=off  SenseTotalForceY=off  SenseTotalForceZ=off  SenseTotalTorque=off  SenseTotalTorqueX=off  SenseTotalTorqueY=off  SenseTotalTorqueZ=off  CompositeWrenchDir=FollowerOnBase  CompositeWrenchFrame=BaseFrame  EquilibriumPosition=0  EquilibriumPositionUnits=deg  SpringStiffness=0  SpringStiffnessUnits=N*m/deg  DampingCoefficient=0  DampingCoefficientUnits=N*m/(deg/s)  TorqueActuationMode=ComputedTorque  MotionActuationMode=InputMotion  SensePosition=on  SenseVelocity=on  SenseAcceleration=on  SenseTorqueForce=on  SenseLowerLimitTorqueForce=off  SenseUpperLimitTorqueForce=off  LowerLimitSpecify=off  LowerLimitBound=-90  LowerLimitBoundUnits=deg  LowerLimitStiffness=1e4  LowerLimitStiffnessUnits=N*m/deg  LowerLimitDamping=10  LowerLimitDampingUnits=N*m/(deg/s)  LowerLimitTransitionRegionWidth=0.1  LowerLimitTransitionRegionWidthUnits=deg  UpperLimitSpecify=off  UpperLimitBound=90  UpperLimitBoundUnits=deg  UpperLimitStiffness=1e4  UpperLimitStiffnessUnits=N*m/deg  UpperLimitDamping=10  UpperLimitDampingUnits=N*m/(deg/s)  UpperLimitTransitionRegionWidth=0.1  UpperLimitTransitionRegionWidthUnits=deg  PositionTargetSpecify=off  PositionTargetPriority=High  PositionTargetValue=0  PositionTargetValueUnits=deg  VelocityTargetSpecify=off  VelocityTargetPriority=High  VelocityTargetValue=0  VelocityTargetValueUnits=deg/s
  Revolute Joint2 : sm_lib/Joints/Revolute Joint  Commented=on  JointMode=Normal  SenseConstraintForce=off  SenseConstraintForceX=off  SenseConstraintForceY=off  SenseConstraintForceZ=off  SenseConstraintTorque=off  SenseConstraintTorqueX=off  SenseConstraintTorqueY=off  SenseConstraintTorqueZ=off  SenseTotalForce=off  SenseTotalForceX=off  SenseTotalForceY=off  SenseTotalForceZ=off  SenseTotalTorque=off  SenseTotalTorqueX=off  SenseTotalTorqueY=off  SenseTotalTorqueZ=off  CompositeWrenchDir=FollowerOnBase  CompositeWrenchFrame=BaseFrame  EquilibriumPosition=0  EquilibriumPositionUnits=deg  SpringStiffness=0  SpringStiffnessUnits=N*m/deg  DampingCoefficient=0  DampingCoefficientUnits=N*m/(deg/s)  TorqueActuationMode=InputTorque  MotionActuationMode=ComputedMotion  SensePosition=on  SenseVelocity=on  SenseAcceleration=on  SenseTorqueForce=on  SenseLowerLimitTorqueForce=off  SenseUpperLimitTorqueForce=off  LowerLimitSpecify=off  LowerLimitBound=-90  LowerLimitBoundUnits=deg  LowerLimitStiffness=1e4  LowerLimitStiffnessUnits=N*m/deg  LowerLimitDamping=10  LowerLimitDampingUnits=N*m/(deg/s)  LowerLimitTransitionRegionWidth=0.1  LowerLimitTransitionRegionWidthUnits=deg  UpperLimitSpecify=off  UpperLimitBound=90  UpperLimitBoundUnits=deg  UpperLimitStiffness=1e4  UpperLimitStiffnessUnits=N*m/deg  UpperLimitDamping=10  UpperLimitDampingUnits=N*m/(deg/s)  UpperLimitTransitionRegionWidth=0.1  UpperLimitTransitionRegionWidthUnits=deg  PositionTargetSpecify=off  PositionTargetPriority=High  PositionTargetValue=0  PositionTargetValueUnits=deg  VelocityTargetSpecify=off  VelocityTargetPriority=High  VelocityTargetValue=0  VelocityTargetValueUnits=deg/s
  Revolute Joint3 : sm_lib/Joints/Revolute Joint  Commented=on  JointMode=Normal  SenseConstraintForce=off  SenseConstraintForceX=off  SenseConstraintForceY=off  SenseConstraintForceZ=off  SenseConstraintTorque=off  SenseConstraintTorqueX=off  SenseConstraintTorqueY=off  SenseConstraintTorqueZ=off  SenseTotalForce=off  SenseTotalForceX=off  SenseTotalForceY=off  SenseTotalForceZ=off  SenseTotalTorque=off  SenseTotalTorqueX=off  SenseTotalTorqueY=off  SenseTotalTorqueZ=off  CompositeWrenchDir=FollowerOnBase  CompositeWrenchFrame=BaseFrame  EquilibriumPosition=0  EquilibriumPositionUnits=deg  SpringStiffness=0  SpringStiffnessUnits=N*m/deg  DampingCoefficient=0  DampingCoefficientUnits=N*m/(deg/s)  TorqueActuationMode=InputTorque  MotionActuationMode=ComputedMotion  SensePosition=on  SenseVelocity=on  SenseAcceleration=on  SenseTorqueForce=on  SenseLowerLimitTorqueForce=off  SenseUpperLimitTorqueForce=off  LowerLimitSpecify=off  LowerLimitBound=-90  LowerLimitBoundUnits=deg  LowerLimitStiffness=1e4  LowerLimitStiffnessUnits=N*m/deg  LowerLimitDamping=10  LowerLimitDampingUnits=N*m/(deg/s)  LowerLimitTransitionRegionWidth=0.1  LowerLimitTransitionRegionWidthUnits=deg  UpperLimitSpecify=off  UpperLimitBound=90  UpperLimitBoundUnits=deg  UpperLimitStiffness=1e4  UpperLimitStiffnessUnits=N*m/deg  UpperLimitDamping=10  UpperLimitDampingUnits=N*m/(deg/s)  UpperLimitTransitionRegionWidth=0.1  UpperLimitTransitionRegionWidthUnits=deg  PositionTargetSpecify=off  PositionTargetPriority=High  PositionTargetValue=0  PositionTargetValueUnits=deg  VelocityTargetSpecify=off  VelocityTargetPriority=High  VelocityTargetValue=0  VelocityTargetValueUnits=deg/s
  Revolute Joint4 : sm_lib/Joints/Revolute Joint  Commented=on  JointMode=Normal  SenseConstraintForce=off  SenseConstraintForceX=off  SenseConstraintForceY=off  SenseConstraintForceZ=off  SenseConstraintTorque=off  SenseConstraintTorqueX=off  SenseConstraintTorqueY=off  SenseConstraintTorqueZ=off  SenseTotalForce=off  SenseTotalForceX=off  SenseTotalForceY=off  SenseTotalForceZ=off  SenseTotalTorque=off  SenseTotalTorqueX=off  SenseTotalTorqueY=off  SenseTotalTorqueZ=off  CompositeWrenchDir=FollowerOnBase  CompositeWrenchFrame=BaseFrame  EquilibriumPosition=0  EquilibriumPositionUnits=deg  SpringStiffness=0  SpringStiffnessUnits=N*m/deg  DampingCoefficient=0  DampingCoefficientUnits=N*m/(deg/s)  TorqueActuationMode=ComputedTorque  MotionActuationMode=InputMotion  SensePosition=on  SenseVelocity=on  SenseAcceleration=on  SenseTorqueForce=on  SenseLowerLimitTorqueForce=off  SenseUpperLimitTorqueForce=off  LowerLimitSpecify=off  LowerLimitBound=-90  LowerLimitBoundUnits=deg  LowerLimitStiffness=1e4  LowerLimitStiffnessUnits=N*m/deg  LowerLimitDamping=10  LowerLimitDampingUnits=N*m/(deg/s)  LowerLimitTransitionRegionWidth=0.1  LowerLimitTransitionRegionWidthUnits=deg  UpperLimitSpecify=off  UpperLimitBound=90  UpperLimitBoundUnits=deg  UpperLimitStiffness=1e4  UpperLimitStiffnessUnits=N*m/deg  UpperLimitDamping=10  UpperLimitDampingUnits=N*m/(deg/s)  UpperLimitTransitionRegionWidth=0.1  UpperLimitTransitionRegionWidthUnits=deg  PositionTargetSpecify=off  PositionTargetPriority=High  PositionTargetValue=0  PositionTargetValueUnits=deg  VelocityTargetSpecify=off  VelocityTargetPriority=High  VelocityTargetValue=0  VelocityTargetValueUnits=deg/s
  Revolute Joint5 : sm_lib/Joints/Revolute Joint  Commented=on  JointMode=Normal  SenseConstraintForce=off  SenseConstraintForceX=off  SenseConstraintForceY=off  SenseConstraintForceZ=off  SenseConstraintTorque=off  SenseConstraintTorqueX=off  SenseConstraintTorqueY=off  SenseConstraintTorqueZ=off  SenseTotalForce=off  SenseTotalForceX=off  SenseTotalForceY=off  SenseTotalForceZ=off  SenseTotalTorque=off  SenseTotalTorqueX=off  SenseTotalTorqueY=off  SenseTotalTorqueZ=off  CompositeWrenchDir=FollowerOnBase  CompositeWrenchFrame=FollowerFrame  EquilibriumPosition=0  EquilibriumPositionUnits=deg  SpringStiffness=0  SpringStiffnessUnits=N*m/deg  DampingCoefficient=0  DampingCoefficientUnits=N*m/(deg/s)  TorqueActuationMode=ComputedTorque  MotionActuationMode=InputMotion  SensePosition=on  SenseVelocity=on  SenseAcceleration=on  SenseTorqueForce=on  SenseLowerLimitTorqueForce=off  SenseUpperLimitTorqueForce=off  LowerLimitSpecify=off  LowerLimitBound=-90  LowerLimitBoundUnits=deg  LowerLimitStiffness=1e4  LowerLimitStiffnessUnits=N*m/deg  LowerLimitDamping=10  LowerLimitDampingUnits=N*m/(deg/s)  LowerLimitTransitionRegionWidth=0.1  LowerLimitTransitionRegionWidthUnits=deg  UpperLimitSpecify=off  UpperLimitBound=90  UpperLimitBoundUnits=deg  UpperLimitStiffness=1e4  UpperLimitStiffnessUnits=N*m/deg  UpperLimitDamping=10  UpperLimitDampingUnits=N*m/(deg/s)  UpperLimitTransitionRegionWidth=0.1  UpperLimitTransitionRegionWidthUnits=deg  PositionTargetSpecify=off  PositionTargetPriority=High  PositionTargetValue=0  PositionTargetValueUnits=deg  VelocityTargetSpecify=off  VelocityTargetPriority=High  VelocityTargetValue=0  VelocityTargetValueUnits=deg/s
  Rigid Transform{,4,6,11} (4 alike) : sm_lib/Frames and Transforms/Rigid Transform  Commented=on  TranslationMethod=Cartesian  TranslationStandardOffset=0  TranslationStandardOffsetUnits=m  TranslationStandardAxis=+Z  TranslationCartesianOffset=[0.01 0 0]  TranslationCartesianOffsetUnits=m  TranslationROffset=0  TranslationROffsetUnits=m  TranslationZOffset=0  TranslationZOffsetUnits=m  TranslationThetaOffset=0  TranslationThetaOffsetUnits=deg  RotationMethod=None  RotationAngleUnits=deg  RotationStandardAxis=+Z  RotationAngle=0.0  RotationArbitraryAxis=[0 0 1]  FollAlignAxisA=+X  BaseAlignAxisA=+Y  FollAlignAxisB=+Y  BaseAlignAxisB=+Z  RotationSequenceAxes=FollowerAxes  RotationSequence=XYX  RotationSequenceAngles=[0 0 0]  RotationSequenceAnglesUnits=deg  RotationMatrix=[1 0 0; 0 1 0; 0 0 1]  Quaternion=[1 0 0 0]
  Rigid Transform{1,7,12,16} (4 alike) : sm_lib/Frames and Transforms/Rigid Transform  Commented=on  TranslationMethod=Cartesian  TranslationStandardOffset=0  TranslationStandardOffsetUnits=m  TranslationStandardAxis=+Z  TranslationCartesianOffset=[-0.01 0 0]  TranslationCartesianOffsetUnits=m  TranslationROffset=0  TranslationROffsetUnits=m  TranslationZOffset=0  TranslationZOffsetUnits=m  TranslationThetaOffset=0  TranslationThetaOffsetUnits=deg  RotationMethod=None  RotationAngleUnits=deg  RotationStandardAxis=+Z  RotationAngle=0.0  RotationArbitraryAxis=[0 0 1]  FollAlignAxisA=+X  BaseAlignAxisA=+Y  FollAlignAxisB=+Y  BaseAlignAxisB=+Z  RotationSequenceAxes=FollowerAxes  RotationSequence=XYX  RotationSequenceAngles=[0 0 0]  RotationSequenceAnglesUnits=deg  RotationMatrix=[1 0 0; 0 1 0; 0 0 1]  Quaternion=[1 0 0 0]
  Rigid Transform10 : sm_lib/Frames and Transforms/Rigid Transform  Commented=on  TranslationMethod=Cartesian  TranslationStandardOffset=0  TranslationStandardOffsetUnits=m  TranslationStandardAxis=+Z  TranslationCartesianOffset=[0 Cube_L/2 0]  TranslationCartesianOffsetUnits=m  TranslationROffset=0  TranslationROffsetUnits=m  TranslationZOffset=0  TranslationZOffsetUnits=m  TranslationThetaOffset=0  TranslationThetaOffsetUnits=deg  RotationMethod=RotationSequence  RotationAngleUnits=deg  RotationStandardAxis=+Z  RotationAngle=0.0  RotationArbitraryAxis=[0 0 1]  FollAlignAxisA=+X  BaseAlignAxisA=+Y  FollAlignAxisB=+Y  BaseAlignAxisB=+Z  RotationSequenceAxes=FollowerAxes  RotationSequence=ZYX  RotationSequenceAngles=[0 0 -90]  RotationSequenceAnglesUnits=deg  RotationMatrix=[1 0 0; 0 1 0; 0 0 1]  Quaternion=[1 0 0 0]
  Rigid Transform{2,8,13,18} (4 alike) : sm_lib/Frames and Transforms/Rigid Transform  Commented=on  TranslationMethod=Cartesian  TranslationStandardOffset=0  TranslationStandardOffsetUnits=m  TranslationStandardAxis=+Z  TranslationCartesianOffset=[0 0.01 0]  TranslationCartesianOffsetUnits=m  TranslationROffset=0  TranslationROffsetUnits=m  TranslationZOffset=0  TranslationZOffsetUnits=m  TranslationThetaOffset=0  TranslationThetaOffsetUnits=deg  RotationMethod=None  RotationAngleUnits=deg  RotationStandardAxis=+Z  RotationAngle=0.0  RotationArbitraryAxis=[0 0 1]  FollAlignAxisA=+X  BaseAlignAxisA=+Y  FollAlignAxisB=+Y  BaseAlignAxisB=+Z  RotationSequenceAxes=FollowerAxes  RotationSequence=XYX  RotationSequenceAngles=[0 0 0]  RotationSequenceAnglesUnits=deg  RotationMatrix=[1 0 0; 0 1 0; 0 0 1]  Quaternion=[1 0 0 0]
  Rigid Transform{3,9,14,19} (4 alike) : sm_lib/Frames and Transforms/Rigid Transform  Commented=on  TranslationMethod=Cartesian  TranslationStandardOffset=0  TranslationStandardOffsetUnits=m  TranslationStandardAxis=+Z  TranslationCartesianOffset=[0 -0.01 0]  TranslationCartesianOffsetUnits=m  TranslationROffset=0  TranslationROffsetUnits=m  TranslationZOffset=0  TranslationZOffsetUnits=m  TranslationThetaOffset=0  TranslationThetaOffsetUnits=deg  RotationMethod=None  RotationAngleUnits=deg  RotationStandardAxis=+Z  RotationAngle=0.0  RotationArbitraryAxis=[0 0 1]  FollAlignAxisA=+X  BaseAlignAxisA=+Y  FollAlignAxisB=+Y  BaseAlignAxisB=+Z  RotationSequenceAxes=FollowerAxes  RotationSequence=XYX  RotationSequenceAngles=[0 0 0]  RotationSequenceAnglesUnits=deg  RotationMatrix=[1 0 0; 0 1 0; 0 0 1]  Quaternion=[1 0 0 0]
  Rigid Transform15 : sm_lib/Frames and Transforms/Rigid Transform  Commented=on  TranslationMethod=Cartesian  TranslationStandardOffset=0  TranslationStandardOffsetUnits=m  TranslationStandardAxis=+Z  TranslationCartesianOffset=[0 0 Cube_L/2]  TranslationCartesianOffsetUnits=m  TranslationROffset=0  TranslationROffsetUnits=m  TranslationZOffset=0  TranslationZOffsetUnits=m  TranslationThetaOffset=0  TranslationThetaOffsetUnits=deg  RotationMethod=None  RotationAngleUnits=deg  RotationStandardAxis=+Z  RotationAngle=0.0  RotationArbitraryAxis=[0 0 1]  FollAlignAxisA=+X  BaseAlignAxisA=+Y  FollAlignAxisB=+Y  BaseAlignAxisB=+Z  RotationSequenceAxes=FollowerAxes  RotationSequence=ZYX  RotationSequenceAngles=[0 90 0]  RotationSequenceAnglesUnits=deg  RotationMatrix=[1 0 0; 0 1 0; 0 0 1]  Quaternion=[1 0 0 0]
  Rigid Transform17 : sm_lib/Frames and Transforms/Rigid Transform  Commented=on  TranslationMethod=Cartesian  TranslationStandardOffset=0  TranslationStandardOffsetUnits=m  TranslationStandardAxis=+Z  TranslationCartesianOffset=[0 0 Cube_L/2]  TranslationCartesianOffsetUnits=m  TranslationROffset=0  TranslationROffsetUnits=m  TranslationZOffset=0  TranslationZOffsetUnits=m  TranslationThetaOffset=0  TranslationThetaOffsetUnits=deg  RotationMethod=None  RotationAngleUnits=deg  RotationStandardAxis=+Z  RotationAngle=0.0  RotationArbitraryAxis=[0 0 1]  FollAlignAxisA=+X  BaseAlignAxisA=+Y  FollAlignAxisB=+Y  BaseAlignAxisB=+Z  RotationSequenceAxes=FollowerAxes  RotationSequence=ZYX  RotationSequenceAngles=[0 90 0]  RotationSequenceAnglesUnits=deg  RotationMatrix=[1 0 0; 0 1 0; 0 0 1]  Quaternion=[1 0 0 0]
  Rigid Transform20 : sm_lib/Frames and Transforms/Rigid Transform  Commented=on  TranslationMethod=Cartesian  TranslationStandardOffset=0  TranslationStandardOffsetUnits=m  TranslationStandardAxis=+Z  TranslationCartesianOffset=[0 0 Cube_L/2]  TranslationCartesianOffsetUnits=m  TranslationROffset=0  TranslationROffsetUnits=m  TranslationZOffset=0  TranslationZOffsetUnits=m  TranslationThetaOffset=0  TranslationThetaOffsetUnits=deg  RotationMethod=None  RotationAngleUnits=deg  RotationStandardAxis=+Z  RotationAngle=0.0  RotationArbitraryAxis=[0 0 1]  FollAlignAxisA=+X  BaseAlignAxisA=+Y  FollAlignAxisB=+Y  BaseAlignAxisB=+Z  RotationSequenceAxes=FollowerAxes  RotationSequence=XYX  RotationSequenceAngles=[0 0 0]  RotationSequenceAnglesUnits=deg  RotationMatrix=[1 0 0; 0 1 0; 0 0 1]  Quaternion=[1 0 0 0]
  Rigid Transform5 : sm_lib/Frames and Transforms/Rigid Transform  Commented=on  TranslationMethod=Cartesian  TranslationStandardOffset=0  TranslationStandardOffsetUnits=m  TranslationStandardAxis=+Z  TranslationCartesianOffset=[Cube_L/2 0 0]  TranslationCartesianOffsetUnits=m  TranslationROffset=0  TranslationROffsetUnits=m  TranslationZOffset=0  TranslationZOffsetUnits=m  TranslationThetaOffset=0  TranslationThetaOffsetUnits=deg  RotationMethod=RotationSequence  RotationAngleUnits=deg  RotationStandardAxis=+Z  RotationAngle=0.0  RotationArbitraryAxis=[0 0 1]  FollAlignAxisA=+X  BaseAlignAxisA=+Y  FollAlignAxisB=+Y  BaseAlignAxisB=+Z  RotationSequenceAxes=FollowerAxes  RotationSequence=ZYX  RotationSequenceAngles=[0 90 0]  RotationSequenceAnglesUnits=deg  RotationMatrix=[1 0 0; 0 1 0; 0 0 1]  Quaternion=[1 0 0 0]
  Rodrigues to Direction Cosine Matrix : Rod2Dcm  Commented=on
  Rotation Angles to Quaternions : sharedtransform/Rotation Angles to Quaternions  rotationOrder=ZYX  aMode=aMode
  Rotation Angles to Quaternions1 : sharedtransform/Rotation Angles to Quaternions  Commented=on  rotationOrder=ZYX  aMode=aMode
  Rotation Angles to Quaternions2 : sharedtransform/Rotation Angles to Quaternions  Commented=on  rotationOrder=ZYX  aMode=aMode
  Scope : Scope  NumInputPorts=3
  Scope{1,4,7..8} (4 alike) : Scope  Commented=on  NumInputPorts=3
  Scope2 : Scope  Commented=on
  Scope3 : Scope  NumInputPorts=3
  Scope5 : Scope  NumInputPorts=3
  Scope6 : Scope  Commented=on
  Selector{,1..5} (6 alike) : Selector  Commented=on  InputPortWidth=3  IndexOptions=Index vector (dialog)  Indices=[3]  OutputSizes=1
  Sim_W : Scope  NumInputPorts=3
  Sim_Wd : Scope  NumInputPorts=3
  Simscape : Scope  Commented=on  NumInputPorts=3
  Simscape_RW : Scope  Commented=on  NumInputPorts=3
  Simscape_Revolute_joint_RW : Scope  Commented=on  NumInputPorts=4
  Simulink-PS Converter{,2,4..5,9..10} (6 alike) : nesl_utility/Simulink-PS Converter  Commented=on  PhysicalDomain=network_engine_domain  SubClassName=ps_input  LeftPortType=input  RightPortType=output  PseudoPeriodic=off  Frequencies=[]  NoiseDistribution=none  NoiseParameters=[]  Unit=1  AffineConversion=off  FilteringAndDerivatives=provide  SimscapeFilterOrder=1  InputFilterTimeConstant=0.001  UdotUserProvided=0
  Simulink-PS Converter1 : nesl_utility/Simulink-PS Converter  PhysicalDomain=network_engine_domain  SubClassName=ps_input  LeftPortType=input  RightPortType=output  PseudoPeriodic=off  Frequencies=[]  NoiseDistribution=none  NoiseParameters=[]  Unit=1  AffineConversion=off  FilteringAndDerivatives=provide  SimscapeFilterOrder=1  InputFilterTimeConstant=0.001  UdotUserProvided=0
  Simulink-PS Converter13 : nesl_utility/Simulink-PS Converter  PhysicalDomain=network_engine_domain  SubClassName=ps_input  LeftPortType=input  RightPortType=output  PseudoPeriodic=off  Frequencies=[]  NoiseDistribution=none  NoiseParameters=[]  Unit=1  AffineConversion=off  FilteringAndDerivatives=provide  SimscapeFilterOrder=1  InputFilterTimeConstant=0.001  UdotUserProvided=2
  Simulink-PS Converter{3,6..8} (4 alike) : nesl_utility/Simulink-PS Converter  Commented=on  PhysicalDomain=network_engine_domain  SubClassName=ps_input  LeftPortType=input  RightPortType=output  PseudoPeriodic=off  Frequencies=[]  NoiseDistribution=none  NoiseParameters=[]  Unit=1  AffineConversion=off  FilteringAndDerivatives=provide  SimscapeFilterOrder=1  InputFilterTimeConstant=0.001  UdotUserProvided=2
  Solver Configuration : nesl_utility/Solver Configuration  Commented=on  PhysicalDomain=network_engine_domain  SubClassName=solver  LeftPortType=input  RightPortType=generic  Tones=[]  Harmonics=[]  SimulateNoise=off  Profile=off  UseLocalSampling=off  EnableSwitchedLinearOptims=on  FrequencyDomain=off  UseCCode=off  RelTol=0.001  AbsTol=0.001  MinStep=1e-09  ToWorkspace=off  RevertToSquareIcSolve=off  NumHomotopyIterations=100  PhasorMode=off  PhasorModeNumHarmonics=1  ConsistencySolver=NEWTON_XTOL_AFTER_FTOL  IndexReductionMethod=DerivativeReplacement  DoDC=off  ResidualTolerance=1e-09  ConsistencyTolSource=GLOBAL  ConsistencyAbsTol=0.001  ConsistencyRelTol=0.001  ConsistencyTolFactor=0.001  UseLocalSolver=off  LocalSolverChoice=NE_BACKWARD_EULER_ADVANCER  ResolveIndetEquations=on  FunctionEvalNumThread=1  LocalSolverSampleTime=0.001  DoFixedCost=off  MaxNonlinIter=3  MaxModeIter=2  ComputeImpulses=off  ImpulseIterations=2  LinearAlgebra=auto  LinearAlgebraNumThread=0  EquationFormulation=NE_TIME_EF  DelaysMemoryBudget=1024  AutomaticFiltering=on  FilteringTimeConstant=0.001  PartitionStorageMethod=AS_NEEDED  PartitionMemoryBudget=1024  PartitionMethod=ROBUST  MultibodyUseLocalSolver=off  MultibodyLocalSolverChoice=ODE1  MultibodyLocalSolverSampleTime=0.001
  Solver Configuration1 : nesl_utility/Solver Configuration  PhysicalDomain=network_engine_domain  SubClassName=solver  LeftPortType=input  RightPortType=generic  Tones=[]  Harmonics=[]  SimulateNoise=off  Profile=off  UseLocalSampling=off  EnableSwitchedLinearOptims=on  FrequencyDomain=off  UseCCode=off  RelTol=0.001  AbsTol=0.001  MinStep=1e-09  ToWorkspace=off  RevertToSquareIcSolve=off  NumHomotopyIterations=100  PhasorMode=off  PhasorModeNumHarmonics=1  ConsistencySolver=NEWTON_XTOL_AFTER_FTOL  IndexReductionMethod=DerivativeReplacement  DoDC=off  ResidualTolerance=1e-09  ConsistencyTolSource=GLOBAL  ConsistencyAbsTol=0.001  ConsistencyRelTol=0.001  ConsistencyTolFactor=0.001  UseLocalSolver=off  LocalSolverChoice=NE_BACKWARD_EULER_ADVANCER  ResolveIndetEquations=on  FunctionEvalNumThread=1  LocalSolverSampleTime=0.001  DoFixedCost=off  MaxNonlinIter=3  MaxModeIter=2  ComputeImpulses=off  ImpulseIterations=2  LinearAlgebra=auto  LinearAlgebraNumThread=0  EquationFormulation=NE_TIME_EF  DelaysMemoryBudget=1024  AutomaticFiltering=on  FilteringTimeConstant=0.001  PartitionStorageMethod=AS_NEEDED  PartitionMemoryBudget=1024  PartitionMethod=ROBUST  MultibodyUseLocalSolver=off  MultibodyLocalSolverChoice=ODE1  MultibodyLocalSolverSampleTime=0.001
  Solver Configuration2 : nesl_utility/Solver Configuration  Commented=on  PhysicalDomain=network_engine_domain  SubClassName=solver  LeftPortType=input  RightPortType=generic  Tones=[]  Harmonics=[]  SimulateNoise=off  Profile=off  UseLocalSampling=off  EnableSwitchedLinearOptims=on  FrequencyDomain=off  UseCCode=off  RelTol=0.001  AbsTol=0.001  MinStep=1e-09  ToWorkspace=off  RevertToSquareIcSolve=off  NumHomotopyIterations=100  PhasorMode=off  PhasorModeNumHarmonics=1  ConsistencySolver=NEWTON_XTOL_AFTER_FTOL  IndexReductionMethod=DerivativeReplacement  DoDC=off  ResidualTolerance=1e-09  ConsistencyTolSource=GLOBAL  ConsistencyAbsTol=0.001  ConsistencyRelTol=0.001  ConsistencyTolFactor=0.001  UseLocalSolver=off  LocalSolverChoice=NE_BACKWARD_EULER_ADVANCER  ResolveIndetEquations=on  FunctionEvalNumThread=1  LocalSolverSampleTime=0.001  DoFixedCost=off  MaxNonlinIter=3  MaxModeIter=2  ComputeImpulses=off  ImpulseIterations=2  LinearAlgebra=auto  LinearAlgebraNumThread=0  EquationFormulation=NE_TIME_EF  DelaysMemoryBudget=1024  AutomaticFiltering=on  FilteringTimeConstant=0.001  PartitionStorageMethod=AS_NEEDED  PartitionMemoryBudget=1024  PartitionMethod=ROBUST  MultibodyUseLocalSolver=off  MultibodyLocalSolverChoice=ODE1  MultibodyLocalSolverSampleTime=0.001
  Sticker{1..16} (16 alike) : sm_lib/Body Elements/Cylindrical Solid  Commented=on  GraphicAmbientColor=[0.15 0.15 0.15 1.0]  BasedOnType=Mass  CenterOfMass=[0 0 0]  CenterOfMassUnits=m  GraphicDiffuseColor=[1.0 1.0 0.2]  CylinderLength=0.00001  CylinderLengthUnits=m  CylinderRadius=0.003  CylinderRadiusUnits=m  Density=1000  DensityUnits=kg/m^3  DoExposeReferenceFrame=on  GraphicEmissiveColor=[0.0 0.0 0.0 1.0]  ExportEntireGeometry=off  SerializedFrames=<Frames><Frame><Id>Frame1</Id><Value><Name>Sticker_F</Name><Origin><Source>GeometricFeature</Source><FeatureName>bottom surface</FeatureName></Origin><PrimaryAxis><DefinedDirection>+Z</DefinedDirection><Source>ReferenceFrame</Source><SourceDirection>+Z</SourceDirection><FeatureName></FeatureName></PrimaryAxis><SecondaryAxis><DefinedDirection>+X</DefinedDirection><Source>ReferenceFrame</Source><SourceDirection>+X</SourceDirection><FeatureName></FeatureName></SecondaryAxis></Value></Frame></Frames>  MarkerShape=Sphere  MarkerSize=10  GraphicType=FromGeometry  InertiaType=CalculateFromGeometry  Mass=0.000000000000000000000000000000000000000000000000000000000000000001  MassUnits=kg  MomentsOfInertia=[1 1 1]  MomentsOfInertiaUnits=kg*m^2  GraphicOpacity=1.0  ProductsOfInertia=[0 0 0]  ProductsOfInertiaUnits=kg*m^2  GraphicShininess=75  GraphicSpecularColor=[0.5 0.5 0.5 1.0]  GraphicVisPropType=SimpleVisualProperties
  Sum{,1..3} (4 alike) : Sum  Inputs=|+-
  Sum5 : Sum  Commented=on  Inputs=|+-
  Transform Sensor : sm_lib/Frames and Transforms/Transform Sensor  MeasurementFrame=Follower  RotationSequence=ZYX  SenseAngle=off  SenseAxis=off  SenseQ=on  SenseR=off  SenseRotationSequence=off  SenseOmegaX=off  SenseOmegaY=off  SenseOmegaZ=off  SenseOmega=on  SenseQDot=off  SenseRDot=off  SenseRotationSequenceDot=off  SenseAlphaX=off  SenseAlphaY=off  SenseAlphaZ=off  SenseAlpha=on  SenseQDDot=off  SenseRDDot=off  SenseX=off  SenseY=off  SenseZ=off  SenseXYZ=off  SenseRad=off  SenseAzim=off  SenseDist=off  SenseInc=off  SenseXDot=off  SenseYDot=off  SenseZDot=off  SenseXYZDot=off  SenseRadDot=off  SenseAzimDot=off  SenseDistDot=off  SenseIncDot=off  SenseXDDot=off  SenseYDDot=off  SenseZDDot=off  SenseXYZDDot=off  SenseRadDDot=off  SenseAzimDDot=off  SenseDistDDot=off  SenseIncDDot=off
  Transform Sensor{1..2,5,7} (4 alike) : sm_lib/Frames and Transforms/Transform Sensor  Commented=on  MeasurementFrame=Follower  RotationSequence=ZYX  SenseAngle=off  SenseAxis=off  SenseQ=on  SenseR=off  SenseRotationSequence=off  SenseOmegaX=off  SenseOmegaY=off  SenseOmegaZ=off  SenseOmega=on  SenseQDot=off  SenseRDot=off  SenseRotationSequenceDot=off  SenseAlphaX=off  SenseAlphaY=off  SenseAlphaZ=off  SenseAlpha=on  SenseQDDot=off  SenseRDDot=off  SenseX=off  SenseY=off  SenseZ=off  SenseXYZ=off  SenseRad=off  SenseAzim=off  SenseDist=off  SenseInc=off  SenseXDot=off  SenseYDot=off  SenseZDot=off  SenseXYZDot=off  SenseRadDot=off  SenseAzimDot=off  SenseDistDot=off  SenseIncDot=off  SenseXDDot=off  SenseYDDot=off  SenseZDDot=off  SenseXYZDDot=off  SenseRadDDot=off  SenseAzimDDot=off  SenseDistDDot=off  SenseIncDDot=off
  Transform Sensor3 : sm_lib/Frames and Transforms/Transform Sensor  Commented=on  MeasurementFrame=World  RotationSequence=ZYX  SenseAngle=off  SenseAxis=off  SenseQ=on  SenseR=off  SenseRotationSequence=off  SenseOmegaX=off  SenseOmegaY=off  SenseOmegaZ=off  SenseOmega=on  SenseQDot=off  SenseRDot=off  SenseRotationSequenceDot=off  SenseAlphaX=off  SenseAlphaY=off  SenseAlphaZ=off  SenseAlpha=on  SenseQDDot=off  SenseRDDot=off  SenseX=off  SenseY=off  SenseZ=off  SenseXYZ=off  SenseRad=off  SenseAzim=off  SenseDist=off  SenseInc=off  SenseXDot=off  SenseYDot=off  SenseZDot=off  SenseXYZDot=off  SenseRadDot=off  SenseAzimDot=off  SenseDistDot=off  SenseIncDot=off  SenseXDDot=off  SenseYDDot=off  SenseZDDot=off  SenseXYZDDot=off  SenseRadDDot=off  SenseAzimDDot=off  SenseDistDDot=off  SenseIncDDot=off
  Transform Sensor4 : sm_lib/Frames and Transforms/Transform Sensor  Commented=on  MeasurementFrame=World  RotationSequence=ZYX  SenseAngle=off  SenseAxis=off  SenseQ=on  SenseR=off  SenseRotationSequence=off  SenseOmegaX=off  SenseOmegaY=off  SenseOmegaZ=off  SenseOmega=on  SenseQDot=off  SenseRDot=off  SenseRotationSequenceDot=off  SenseAlphaX=off  SenseAlphaY=off  SenseAlphaZ=off  SenseAlpha=on  SenseQDDot=off  SenseRDDot=off  SenseX=off  SenseY=off  SenseZ=off  SenseXYZ=off  SenseRad=off  SenseAzim=off  SenseDist=off  SenseInc=off  SenseXDot=off  SenseYDot=off  SenseZDot=off  SenseXYZDot=off  SenseRadDot=off  SenseAzimDot=off  SenseDistDot=off  SenseIncDot=off  SenseXDDot=off  SenseYDDot=off  SenseZDDot=off  SenseXYZDDot=off  SenseRadDDot=off  SenseAzimDDot=off  SenseDistDDot=off  SenseIncDDot=off
  Transform Sensor6 : sm_lib/Frames and Transforms/Transform Sensor  Commented=on  MeasurementFrame=World  RotationSequence=ZYX  SenseAngle=off  SenseAxis=off  SenseQ=on  SenseR=off  SenseRotationSequence=off  SenseOmegaX=off  SenseOmegaY=off  SenseOmegaZ=off  SenseOmega=on  SenseQDot=off  SenseRDot=off  SenseRotationSequenceDot=off  SenseAlphaX=off  SenseAlphaY=off  SenseAlphaZ=off  SenseAlpha=on  SenseQDDot=off  SenseRDDot=off  SenseX=off  SenseY=off  SenseZ=off  SenseXYZ=off  SenseRad=off  SenseAzim=off  SenseDist=off  SenseInc=off  SenseXDot=off  SenseYDot=off  SenseZDot=off  SenseXYZDot=off  SenseRadDot=off  SenseAzimDot=off  SenseDistDot=off  SenseIncDot=off  SenseXDDot=off  SenseYDDot=off  SenseZDDot=off  SenseXYZDDot=off  SenseRadDDot=off  SenseAzimDDot=off  SenseDistDDot=off  SenseIncDDot=off
  Universal Joint : sm_lib/Joints/Universal Joint  JointMode=Normal  SenseConstraintForce=off  SenseConstraintForceX=off  SenseConstraintForceY=off  SenseConstraintForceZ=off  SenseConstraintTorque=off  SenseConstraintTorqueX=off  SenseConstraintTorqueY=off  SenseConstraintTorqueZ=off  SenseTotalForce=off  SenseTotalForceX=off  SenseTotalForceY=off  SenseTotalForceZ=off  SenseTotalTorque=off  SenseTotalTorqueX=off  SenseTotalTorqueY=off  SenseTotalTorqueZ=off  CompositeWrenchDir=FollowerOnBase  CompositeWrenchFrame=BaseFrame  RxEquilibriumPosition=0  RxEquilibriumPositionUnits=deg  RxSpringStiffness=0  RxSpringStiffnessUnits=N*m/deg  RxDampingCoefficient=0  RxDampingCoefficientUnits=N*m/(deg/s)  RxTorqueActuationMode=ComputedTorque  RxMotionActuationMode=InputMotion  RxSensePosition=off  RxSenseVelocity=off  RxSenseAcceleration=off  RxSenseTorqueForce=off  RxSenseLowerLimitTorqueForce=off  RxSenseUpperLimitTorqueForce=off  RxLowerLimitSpecify=off  RxLowerLimitBound=-90  RxLowerLimitBoundUnits=deg  RxLowerLimitStiffness=1e4  RxLowerLimitStiffnessUnits=N*m/deg  RxLowerLimitDamping=10  RxLowerLimitDampingUnits=N*m/(deg/s)  RxLowerLimitTransitionRegionWidth=0.1  RxLowerLimitTransitionRegionWidthUnits=deg  RxUpperLimitSpecify=off  RxUpperLimitBound=90  RxUpperLimitBoundUnits=deg  RxUpperLimitStiffness=1e4  RxUpperLimitStiffnessUnits=N*m/deg  RxUpperLimitDamping=10  RxUpperLimitDampingUnits=N*m/(deg/s)  RxUpperLimitTransitionRegionWidth=0.1  RxUpperLimitTransitionRegionWidthUnits=deg  RxPositionTargetSpecify=off  RxPositionTargetPriority=High  RxPositionTargetValue=0  RxPositionTargetValueUnits=deg  RxVelocityTargetSpecify=off  RxVelocityTargetPriority=High  RxVelocityTargetValue=0  RxVelocityTargetValueUnits=deg/s  RyEquilibriumPosition=0  RyEquilibriumPositionUnits=deg  RySpringStiffness=0  RySpringStiffnessUnits=N*m/deg  RyDampingCoefficient=0  RyDampingCoefficientUnits=N*m/(deg/s)  RyTorqueActuationMode=ComputedTorque  RyMotionActuationMode=InputMotion  RySensePosition=off  RySenseVelocity=off  RySenseAcceleration=off  RySenseTorqueForce=off  RySenseLowerLimitTorqueForce=off  RySenseUpperLimitTorqueForce=off  RyLowerLimitSpecify=off  RyLowerLimitBound=-90  RyLowerLimitBoundUnits=deg  RyLowerLimitStiffness=1e4  RyLowerLimitStiffnessUnits=N*m/deg  RyLowerLimitDamping=10  RyLowerLimitDampingUnits=N*m/(deg/s)  RyLowerLimitTransitionRegionWidth=0.1  RyLowerLimitTransitionRegionWidthUnits=deg  RyUpperLimitSpecify=off  RyUpperLimitBound=90  RyUpperLimitBoundUnits=deg  RyUpperLimitStiffness=1e4  RyUpperLimitStiffnessUnits=N*m/deg  RyUpperLimitDamping=10  RyUpperLimitDampingUnits=N*m/(deg/s)  RyUpperLimitTransitionRegionWidth=0.1  RyUpperLimitTransitionRegionWidthUnits=deg  RyPositionTargetSpecify=off  RyPositionTargetPriority=High  RyPositionTargetValue=0  RyPositionTargetValueUnits=deg  RyVelocityTargetSpecify=off  RyVelocityTargetPriority=High  RyVelocityTargetValue=0  RyVelocityTargetValueUnits=deg/s
  Wheel_Joint_Accel : Goto  Commented=on  GotoTag=RW_Joint_Accel
  Wheel_Joint_Angle : Goto  Commented=on  GotoTag=RW_Joint_Angle
  Wheel_Joint_Rate : Goto  Commented=on  GotoTag=RW_Joint_Rate
  Wheel_joint_Accel rad/s^1 : Constant  Value=0
  Wheel_joint_Accel rad/s^2 : Constant  Commented=on
  Wheel_joint_Accel rad/s^3 : Constant
  World Frame : sm_lib/Frames and Transforms/World Frame  Commented=on
  World Frame1 : sm_lib/Frames and Transforms/World Frame
  World Frame2 : sm_lib/Frames and Transforms/World Frame  Commented=on
  angle_differ_differ : Scope
  angle_differ_myfunc : Scope
  deriviation of quaternion1 : MATLAB Function  Commented=on  TreatAsAtomicUnit=on
  deriviation of quaternion2 : MATLAB Function  Commented=on  TreatAsAtomicUnit=on
  diff_angle : MATLAB Function  TreatAsAtomicUnit=on
  quat_diff_to_ZYX : Scope  NumInputPorts=3
  quat_to_ZYX_diff : Scope  NumInputPorts=3
  quaternion to Euler angle 1 : MATLAB Function  Commented=on  TreatAsAtomicUnit=on
  rigid body : MATLAB Function  TreatAsAtomicUnit=on
  rigid body1 : MATLAB Function  TreatAsAtomicUnit=on
  rigid body2 : MATLAB Function  TreatAsAtomicUnit=on
  rigid body3 : MATLAB Function  Commented=on  TreatAsAtomicUnit=on
  rigid body4 : MATLAB Function  Commented=on  TreatAsAtomicUnit=on
  simscape_RW_angle : Scope  Commented=on  NumInputPorts=3
  simscape_RW_w : Scope  Commented=on  NumInputPorts=3
  simscape_angle : Scope  Commented=on  NumInputPorts=3
  simscape_w : Scope  Commented=on  NumInputPorts=3
  w_error : Scope
  wd_error : Scope
  wires:
  rigid body2/1(angle) -> Radians to Degrees4/1
  Demux2/1 -> Scope5/1
  Quaternion Normalize/1 -> rigid body2/1(q), rigid body1/2(q), [Euler_eq_quat]
  Constant1/1 -> Rotation Angles to Quaternions/1
  Radians to Degrees5/1 -> Scope3/3
  Rotation Angles to Quaternions/1 -> Integrator1/2
  rigid body/1(omega_prime) -> [Euler_eq_wd], Display1/1, Radians to Degrees5/1, Integrator/1
  Radians to Degrees4/1 -> Display2/1, Demux2/1, Scope3/1, Sum/2
  Demux2/3 -> Scope5/3
  Integrator1/1 -> Quaternion Normalize/1
  Demux2/2 -> Scope5/2
  Radians to Degrees3/1 -> Scope3/2
  [Torque_ext] -> rigid body/1(t_ext)
  rigid body1/1(q_prime) -> Integrator1/1
  Integrator/1 -> rigid body/2(omega), Radians to Degrees3/1, rigid body1/1(w), [Euler_eq_w]
  Degrees to Radians/1 -> Integrator/2
  Constant2/1 -> Degrees to Radians/1
  Constant3/1 -> [Torque_ext]
  Radians to Degrees/1 -> [Simscape_w], Scope/2
  Radians to Degrees1/1 -> [Simscape_wd], Scope/3
  PS-Simulink Converter/1 -> [Simscape_quat], Quaternions to Rotation Angles/1
  [Torque_ext] -> Simulink-PS Converter1/1
  PS-Simulink Converter2/1 -> Radians to Degrees1/1, Display/1
  PS-Simulink Converter1/1 -> Radians to Degrees/1
  Quaternions to Rotation Angles/1 -> Radians to Degrees2/1
  Radians to Degrees2/1 -> Sum/1, Scope/1
  [Euler_eq_wd] -> Radians to Degrees9/1
  [Euler_eq_quat] -> Quaternion Inverse/1
  [Euler_eq_w] -> Radians to Degrees10/1
  Sum2/1 -> w_error/1
  Radians to Degrees9/1 -> Sum1/2
  [Simscape_wd] -> Sum1/1
  [Simscape_w] -> Sum2/1
  Quaternion Multiplication/1 -> diff_angle/1(q_err), Quaternions to Rotation Angles3/1
  Sum1/1 -> wd_error/1
  Quaternion Inverse/1 -> Quaternion Multiplication/2
  Quaternions to Rotation Angles3/1 -> Radians to Degrees6/1
  Radians to Degrees10/1 -> Sum2/2
  [Simscape_quat] -> Quaternion Multiplication/1
  Demux/2 -> quat_to_ZYX_diff/2
  Sum/1 -> Demux/1
  Demux/1 -> Sum3/1, quat_to_ZYX_diff/1
  Demux/3 -> quat_to_ZYX_diff/3
  Radians to Degrees6/1 -> Demux1/1
  Sum3/1 -> angle_differ_differ/1
  Demux1/1 -> quat_diff_to_ZYX/1, Sum3/2
  Demux1/2 -> quat_diff_to_ZYX/2
  Demux1/3 -> quat_diff_to_ZYX/3
  diff_angle/1(angle_err) -> Radians to Degrees7/1
  Radians to Degrees7/1 -> angle_differ_myfunc/1
  PS-Simulink Converter23/1 -> Goto32/1
  From18/1 -> Simscape_Revolute_joint_RW/2
  Demux5/1 -> simscape_RW_w/1
  Demux5/3 -> simscape_RW_w/3
  Demux6/3 -> simscape_w/3
  Demux6/1 -> simscape_w/1
  PS-Simulink Converter25/1 -> Goto31/1
  From11/1 -> Simscape_Revolute_joint_RW/4
  From43/1 -> Demux5/1, Simscape_RW/2
  Demux4/2 -> Simulink-PS Converter5/1
  From13/1 -> Demux10/1
  From16/1 -> Simscape_Revolute_joint_RW/1
  Constant5/1 -> Goto34/1
  From9/1 -> Demux6/1, Simscape/2
  PS-Simulink Converter24/1 -> Goto37/1
  From19/1 -> Simscape_Revolute_joint_RW/3
  From38/1 -> rigid body3/2(t_ext)
  Demux23/2 -> simscape_RW_angle/2
  Demux23/1 -> simscape_RW_angle/1
  Demux23/3 -> simscape_RW_angle/3
  PS-Simulink Converter26/1 -> Goto14/1
  Quaternions to Rotation Angles2/1 -> Radians to Degrees14/1
  Radians to Degrees13/1 -> Goto13/1
  Demux7/3 -> simscape_angle/3
  PS-Simulink Converter5/1 -> Goto7/1
  Constant6/1 -> Goto36/1
  From12/1 -> Demux7/1, Simscape/1
  quaternion to Euler angle 1/1(angle) -> Radians to Degrees12/1
  Quaternion Normalize2/1 -> quaternion to Euler angle 1/1(q), deriviation of quaternion2/2(q)
  Demux24/2 -> Scope4/2
  deriviation of quaternion2/1(q_prime) -> Integrator7/1
  Demux24/1 -> Sum5/2, Scope4/1
  Rotation Angles to Quaternions2/1 -> Integrator7/2
  rigid body3/1(omega_prime) -> Add1/2, Integrator4/1
  Integrator5/1 -> Integrator6/1, Simulink-PS Converter3/2
  Radians to Degrees12/1 -> Demux24/1
  From40/1 -> Add1/1
  Integrator6/1 -> Simulink-PS Converter3/1
  Degrees to Radians2/1 -> Integrator4/2
  Sum5/1 -> Scope6/1
  From41/1 -> Demux25/1
  PS-Simulink Converter12/1 -> Goto33/1
  PS-Simulink Converter27/1 -> Goto15/1
  From17/1 -> Simulink-PS Converter2/1
  PS-Simulink Converter28/1 -> rigid body3/1(Ib), Display3/1
  PS-Simulink Converter3/1 -> Goto35/1
  Add/1 -> Scope1/3
  PS-Simulink Converter9/1 -> Goto18/1, Quaternions to Rotation Angles2/1
  Radians to Degrees11/1 -> Goto27/1
  PS-Simulink Converter17/1 -> Goto24/1
  From47/1 -> rigid body3/5(omega_rw_prime)
  Quaternions to Rotation Angles5/1 -> Radians to Degrees11/1
  From39/1 -> Scope1/2, Add/2
  Integrator7/1 -> Quaternion Normalize2/1
  PS-Simulink Converter20/1 -> Goto28/1, Quaternions to Rotation Angles5/1
  PS-Simulink Converter21/1 -> Goto25/1
  PS-Simulink Converter19/1 -> Goto29/1
  Quaternions to Rotation Angles4/1 -> Radians to Degrees8/1
  Demux5/2 -> simscape_RW_w/2
  From15/1 -> Demux4/1
  Constant7/1 -> Degrees to Radians2/1
  PS-Simulink Converter10/1 -> Goto8/1, Display4/1
  PS-Simulink Converter6/1 -> Goto19/1, Quaternions to Rotation Angles1/1
  Constant8/1 -> Integrator5/1, Simulink-PS Converter3/3
  PS-Simulink Converter8/1 -> Goto12/1
  Radians to Degrees8/1 -> Goto22/1
  Demux24/3 -> Scope4/3
  From42/1 -> Demux23/1, Simscape_RW/1
  Demux25/1 -> Sum5/1
  Demux7/1 -> simscape_angle/1
  Quaternions to Rotation Angles1/1 -> Radians to Degrees13/1
  Demux3/1 -> Simulink-PS Converter4/1
  Add1/1 -> Scope2/1
  PS-Simulink Converter18/1 -> Goto30/1
  Demux6/2 -> simscape_w/2
  From14/1 -> Demux3/1
  PS-Simulink Converter15/1 -> Goto17/1
  Demux7/2 -> simscape_angle/2
  Demux10/3 -> Simulink-PS Converter/1
  PS-Simulink Converter16/1 -> Goto21/1
  (rad/sec) to RPM4/1 -> Scope1/1
  PS-Simulink Converter14/1 -> Goto23/1, Quaternions to Rotation Angles4/1
  Integrator4/1 -> rigid body3/3(omega), (rad/sec) to RPM4/1, deriviation of quaternion2/1(w), Add/1
  PS-Simulink Converter7/1 -> Goto11/1
  Radians to Degrees14/1 -> Goto16/1
  PS-Simulink Converter11/1 -> Goto10/1
  From44/1 -> Simscape_RW/3
  From46/1 -> rigid body3/4(omega_rw)
  Constant9/1 -> Rotation Angles to Quaternions2/1
  PS-Simulink Converter13/1 -> Goto9/1
  From10/1 -> Simscape/3
  PS-Simulink Converter4/1 -> Goto20/1
  PS-Simulink Converter22/1 -> Goto26/1
  Constant10/1 -> Integrator2/1, Simulink-PS Converter6/3
  Integrator3/1 -> Simulink-PS Converter6/1
  Integrator2/1 -> Integrator3/1, Simulink-PS Converter6/2
  Integrator8/1 -> Integrator9/1, Simulink-PS Converter7/2
  Integrator9/1 -> Simulink-PS Converter7/1
  Constant11/1 -> Integrator8/1, Simulink-PS Converter7/3
  Add4/1 -> "RW_diff(Sim,Rev) : wd, w"/2
  Constant12/1 -> Mux4/2, Mux5/1, Mux5/2, Mux4/1
  PS-Simulink Converter35/1 -> Display10/1
  Selector4/1 -> Divide/1
  From32/1 -> Selector4/1
  From35/1 -> Mux2/3
  From33/1 -> Divide/2
  Selector3/1 -> Mux1/3
  PS-Simulink Converter38/1 -> Goto55/1
  Degrees to Radians1/1 -> Integrator12/2
  From25/1 -> Selector2/1
  Selector/1 -> Add4/1
  From/1 -> Mux4/3
  Divide/1 -> Display9/1
  Integrator13/1 -> Quaternion Normalize1/1
  Radians to Degrees18/1 -> "ERROR : Wd, W, Quat"/1
  Selector2/1 -> Mux/3
  From24/1 -> rigid body4/1(Wheel_MOI)
  PS-Simulink Converter30/1 -> Goto48/1
  Selector1/1 -> Add5/1
  From52/1 -> Simulink-PS Converter8/1
  From31/1 -> Selector1/1
  From49/1 -> Mux5/3
  From20/1 -> Selector/1
  PS-Simulink Converter37/1 -> Goto54/1
  From37/1 -> Add4/2
  From48/1 -> Add5/2
  PS-Simulink Converter36/1 -> Goto39/1
  PS-Simulink Converter39/1 -> Goto40/1
  From23/1 -> Quaternion Multiplication1/1
  Mux1/1 -> Reshape1/1
  PS-Simulink Converter32/1 -> Goto41/1
  Radians to Degrees16/1 -> "ERROR : Wd, W, Quat"/2
  Quaternions to Rotation Angles6/1 -> Radians to Degrees15/1
  From22/1 -> Quaternion Inverse1/1
  From29/1 -> Add2/2
  Radians to Degrees15/1 -> "ERROR : Wd, W, Quat"/3
  Add3/1 -> Radians to Degrees16/1
  From21/1 -> Add3/1
  Quaternion Multiplication1/1 -> Quaternions to Rotation Angles6/1
  Add2/1 -> Radians to Degrees18/1
  Integrator12/1 -> deriviation of quaternion1/1(w), rigid body4/4(omega), Goto49/1
  From53/1 -> Add2/1
  From36/1 -> Mux3/3
  Rotation Angles to Quaternions1/1 -> Integrator13/2
  Integrator10/1 -> Integrator11/1, Wheel_Joint_Rate/1
  From51/1 -> Simulink-PS Converter8/2
  From50/1 -> Simulink-PS Converter8/3
  From26/1 -> rigid body4/2(Ib)
  Wheel_joint_Accel rad/s^2/1 -> Wheel_Joint_Accel/1, Integrator10/1
  Quaternion Inverse1/1 -> Quaternion Multiplication1/2
  From27/1 -> Add3/2
  PS-Simulink Converter31/1 -> Goto47/1, Display6/1
  Constant14/1 -> Gain/1
  Constant17/1 -> Rotation Angles to Quaternions1/1
  Gain/1 -> Goto52/1
  PS-Simulink Converter40/1 -> Goto46/1, Quaternions to Rotation Angles7/1
  From45/1 -> rigid body4/3(t_ext)
  Quaternion Normalize1/1 -> Goto50/1, deriviation of quaternion1/2(q)
  PS-Simulink Converter42/1 -> Goto44/1
  Integrator11/1 -> Wheel_Joint_Angle/1
  rigid body4/1(omega_prime) -> Integrator12/1, Goto38/1
  deriviation of quaternion1/1(q_prime) -> Integrator13/1
  Mux5/1 -> Reshape5/1
  PS-Simulink Converter29/1 -> Goto53/1
  Quaternions to Rotation Angles7/1 -> Radians to Degrees17/1
  From28/1 -> Simulink-PS Converter9/1
  Constant16/1 -> Degrees to Radians1/1
  Add5/1 -> "RW_diff(Sim,Rev) : wd, w"/1
  Radians to Degrees17/1 -> Goto45/1
  Mux4/1 -> Reshape4/1
  Constant15/1 -> Goto42/1
  Mux2/1 -> Reshape2/1
  PS-Simulink Converter43/1 -> Display5/1
  PS-Simulink Converter41/1 -> Goto43/1
  Selector5/1 -> Simulink-PS Converter10/1
  PS-Simulink Converter33/1 -> Display7/1
  PS-Simulink Converter34/1 -> Goto51/1, Display8/1
  Constant/1 -> Mux2/2, Mux3/1, Mux3/2, Mux2/1
  Constant13/1 -> Mux1/2, Mux1/1, Mux/2, Mux/1
  Mux3/1 -> Reshape3/1
  From34/1 -> Selector5/1
  From30/1 -> Selector3/1
  Mux/1 -> Reshape/1
  Demux8/1 -> Scope7/1
  Demux8/2 -> Scope7/2
  Demux8/3 -> Scope7/3
  From54/1 -> Demux8/1
  Demux9/3 -> Scope8/3
  Demux9/2 -> Scope8/2
  From55/1 -> Demux9/1
  Demux9/1 -> Scope8/1
  Reshape2/1 -> rigid body4/5(omega_rw)
  Reshape3/1 -> rigid body4/6(omega_rw_prime)
  [Simscape_w] -> Degrees to Radians3/1
  Demux11/1 -> Sim_W/1
  Demux11/2 -> Sim_W/2
  Demux11/3 -> Sim_W/3
  [Simscape_wd] -> Degrees to Radians4/1
  Demux12/1 -> Sim_Wd/1
  Demux12/2 -> Sim_Wd/2
  Demux12/3 -> Sim_Wd/3
  Integrator15/1 -> [RW_Joint_Angle]
  Wheel_joint_Accel rad/s^1/1 -> [RW_Joint_Accel]
  Wheel_joint_Accel rad/s^3/1 -> Integrator15/1, [RW_Joint_Rate]
  Degrees to Radians3/1 -> Demux11/1
  Degrees to Radians4/1 -> Demux12/1
  [RW_Joint_Rate] -> Simulink-PS Converter13/2
  [RW_Joint_Accel] -> Simulink-PS Converter13/3
  [RW_Joint_Angle] -> Simulink-PS Converter13/1
  connections:
  Solver Configuration1/RConn1 -- World Frame1/RConn1 -- Universal Joint/LConn1 -- Transform Sensor/LConn1 -- Mechanism Configuration1/RConn1
  Transform Sensor/RConn1 -- Base/LConn1 -- External Force and Torque/RConn1
  Transform Sensor/RConn2 -- PS-Simulink Converter/LConn1
  Simulink-PS Converter1/RConn1 -- External Force and Torque/LConn1
  PS-Simulink Converter1/LConn1 -- Transform Sensor/RConn3
  Universal Joint/RConn1 -- Base/RConn1
  PS-Simulink Converter2/LConn1 -- Transform Sensor/RConn4
  External Force and Torque1/RConn1 -- Inertia Sensor/LConn1 -- Transform Sensor2/RConn1 -- Rigid Transform5/LConn1 -- Rigid Transform15/LConn1 -- Rigid Transform10/LConn1 -- Base1/LConn1
  Rigid Transform2/LConn1 -- Rigid Transform1/LConn1 -- Fly_Wheel_Z/LConn1 -- Inertia Sensor1/LConn1 -- Rigid Transform/LConn1 -- Rigid Transform3/LConn1
  Revolute Joint2/RConn1 -- Fly_Wheel_X/RConn1 -- Transform Sensor3/RConn1
  Rigid Transform8/LConn1 -- Rigid Transform6/LConn1 -- Fly_Wheel_X/LConn1 -- Rigid Transform7/LConn1 -- Rigid Transform9/LConn1
  Rigid Transform13/LConn1 -- Rigid Transform14/LConn1 -- Rigid Transform11/LConn1 -- Fly_Wheel_Y/LConn1 -- Rigid Transform12/LConn1
  Fly_Wheel_Z/RConn1 -- Revolute Joint/RConn1 -- Transform Sensor1/RConn1
  Revolute Joint3/RConn1 -- Fly_Wheel_Y/RConn1 -- Transform Sensor4/RConn1
  Mechanism Configuration/RConn1 -- Solver Configuration/RConn1 -- 6-DOF Joint/LConn1 -- World Frame/RConn1
  PS-Simulink Converter18/LConn1 -- Revolute Joint3/RConn3
  PS-Simulink Converter11/LConn1 -- Revolute Joint2/RConn2
  Revolute Joint3/RConn4 -- PS-Simulink Converter19/LConn1
  Transform Sensor2/RConn4 -- PS-Simulink Converter27/LConn1
  Sticker7/LConn1 -- Rigid Transform8/RConn1
  PS-Simulink Converter3/LConn1 -- Revolute Joint/RConn2
  Sticker2/LConn1 -- Rigid Transform1/RConn1
  Sticker10/LConn1 -- Rigid Transform12/RConn1
  Rigid Transform11/RConn1 -- Sticker9/LConn1
  PS-Simulink Converter28/LConn1 -- Inertia Sensor/RConn1
  Simulink-PS Converter4/RConn1 -- Revolute Joint2/LConn2
  Revolute Joint2/RConn5 -- PS-Simulink Converter24/LConn1
  Transform Sensor2/RConn2 -- PS-Simulink Converter9/LConn1
  Sticker3/LConn1 -- Rigid Transform2/RConn1
  Simulink-PS Converter3/RConn1 -- Revolute Joint1/LConn2
  Rigid Transform/RConn1 -- Sticker1/LConn1
  PS-Simulink Converter21/LConn1 -- Transform Sensor4/RConn3
  Transform Sensor1/RConn2 -- PS-Simulink Converter6/LConn1
  Sticker12/LConn1 -- Rigid Transform14/RConn1
  Revolute Joint/RConn5 -- PS-Simulink Converter23/LConn1
  PS-Simulink Converter12/LConn1 -- Revolute Joint2/RConn3
  Transform Sensor1/RConn4 -- PS-Simulink Converter8/LConn1
  PS-Simulink Converter26/LConn1 -- Transform Sensor2/RConn3
  Revolute Joint2/RConn4 -- PS-Simulink Converter13/LConn1
  Transform Sensor4/RConn2 -- PS-Simulink Converter20/LConn1
  Rigid Transform6/RConn1 -- Sticker5/LConn1
  Sticker6/LConn1 -- Rigid Transform7/RConn1
  Transform Sensor4/RConn4 -- PS-Simulink Converter22/LConn1
  PS-Simulink Converter17/LConn1 -- Revolute Joint3/RConn2
  PS-Simulink Converter7/LConn1 -- Transform Sensor1/RConn3
  Inertia Sensor1/RConn1 -- PS-Simulink Converter10/LConn1
  6-DOF Joint/RConn1 -- Base1/RConn1
  PS-Simulink Converter4/LConn1 -- Revolute Joint/RConn3
  Sticker8/LConn1 -- Rigid Transform9/RConn1
  Revolute Joint3/RConn5 -- PS-Simulink Converter25/LConn1
  Transform Sensor3/RConn2 -- PS-Simulink Converter14/LConn1
  Simulink-PS Converter5/RConn1 -- Revolute Joint3/LConn2
  Rigid Transform5/RConn1 -- Revolute Joint2/LConn1
  Rigid Transform15/RConn1 -- Revolute Joint/LConn1
  Revolute Joint/RConn4 -- PS-Simulink Converter5/LConn1
  Transform Sensor3/RConn4 -- PS-Simulink Converter16/LConn1
  Simulink-PS Converter2/RConn1 -- External Force and Torque1/LConn1
  Sticker4/LConn1 -- Rigid Transform3/RConn1
  Sticker11/LConn1 -- Rigid Transform13/RConn1
  PS-Simulink Converter15/LConn1 -- Transform Sensor3/RConn3
  Rigid Transform10/RConn1 -- Revolute Joint3/LConn1
  Simulink-PS Converter6/RConn1 -- Revolute Joint4/LConn2
  Simulink-PS Converter7/RConn1 -- Revolute Joint/LConn2
  Rigid Transform20/RConn1 -- Revolute Joint5/LConn1
  Transform Sensor6/RConn1 -- Transform Sensor7/RConn1 -- External Force and Torque2/RConn1 -- Transform Sensor5/LConn1 -- Base2/LConn1 -- Rigid Transform20/LConn1 -- Rigid Transform17/RConn1 -- Inertia Sensor2/LConn1
  Fly_Wheel/LConn1 -- Rigid Transform16/LConn1 -- Rigid Transform19/LConn1 -- Rigid Transform18/LConn1 -- Inertia Sensor3/LConn1 -- Rigid Transform4/LConn1
  Revolute Joint5/RConn1 -- Fly_Wheel/RConn1 -- Transform Sensor5/RConn1
  Inertia Sensor2/RConn2 -- PS-Simulink Converter43/LConn1
  PS-Simulink Converter35/LConn1 -- Inertia Sensor2/RConn1
  Mechanism Configuration2/RConn1 -- Transform Sensor7/LConn1 -- 6-DOF Joint2/LConn1 -- Solver Configuration2/RConn1 -- World Frame2/RConn1
  PS-Simulink Converter30/LConn1 -- Revolute Joint5/RConn3
  Inertia Sensor3/RConn1 -- PS-Simulink Converter31/LConn1
  Sticker15/LConn1 -- Rigid Transform18/RConn1
  PS-Simulink Converter38/LConn1 -- Transform Sensor7/RConn4
  Rigid Transform17/LConn1 -- Inertia Sensor4/LConn1
  Transform Sensor7/RConn3 -- PS-Simulink Converter37/LConn1
  Rigid Transform4/RConn1 -- Sticker13/LConn1
  PS-Simulink Converter34/LConn1 -- Inertia Sensor4/RConn1
  Transform Sensor6/RConn4 -- PS-Simulink Converter42/LConn1
  PS-Simulink Converter32/LConn1 -- Transform Sensor5/RConn4
  Transform Sensor6/RConn2 -- PS-Simulink Converter40/LConn1
  PS-Simulink Converter39/LConn1 -- Transform Sensor5/RConn3
  PS-Simulink Converter29/LConn1 -- Revolute Joint5/RConn2
  Revolute Joint5/RConn5 -- PS-Simulink Converter33/LConn1
  Sticker16/LConn1 -- Rigid Transform19/RConn1
  PS-Simulink Converter41/LConn1 -- Transform Sensor6/RConn3
  Revolute Joint5/RConn4 -- PS-Simulink Converter36/LConn1
  Sticker14/LConn1 -- Rigid Transform16/RConn1
  Simulink-PS Converter9/RConn1 -- External Force and Torque2/LConn1
  Simulink-PS Converter8/RConn1 -- Revolute Joint5/LConn2
  6-DOF Joint2/RConn1 -- Base2/RConn1
  Simulink-PS Converter13/RConn1 -- Universal Joint/LConn3 -- Universal Joint/LConn2
